simulink model "WSCC_Indian_400kV_test1"  (R2021b)
settings: Solver=FixedStepDiscrete  StartTime=0.0  StopTime=1  FixedStep=5e-7  RelTol=1e-3
undefined symbols (not defined in the file or in its folder): D1, Delta
libraries: spsPowerPositiveSequenceLib x24, spsThreePhaseVIMeasurementLib x21, spsFourierLib x18, spsThreePhaseBreakerLib x12, spsDistributedParametersLineLib x12, spsLoadFlowBusLib x9, spsRMSLib x6, spsThreePhaseParallelRLCLoadLib x6, spsSynchronousMachinepuStandardLib x4, spsExcitationSystemLib x3, spsMultiBandPowerSystemStabilizerLib x3, spsSteamTurbineandGovernorLib x3
(part 1 of 2)
settings Model: Creator=MARI  LastModifiedBy=DELL
settings SolverCC: AlgebraicLoopSolver=TrustRegion
settings DataIOCC: SignalLogging=off  DSMLogging=off
settings DebuggingCC: UnconnectedInputMsg=none  UnconnectedOutputMsg=none  UnconnectedLineMsg=none  SFMachineParentedDataDiag=warning  ArithmeticOperatorsInVariantConditions=warning
settings SFSimCC: SimUseLocalCustomCode=off  CustomCodeUndefinedFunction=UseInterfaceOnly
settings RTWCC: RTWUseLocalCustomCode=off

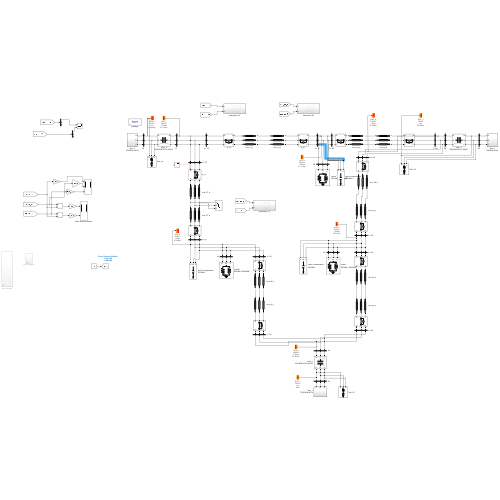
[thumbnail: Simulink's stored preview of the top-level diagram]
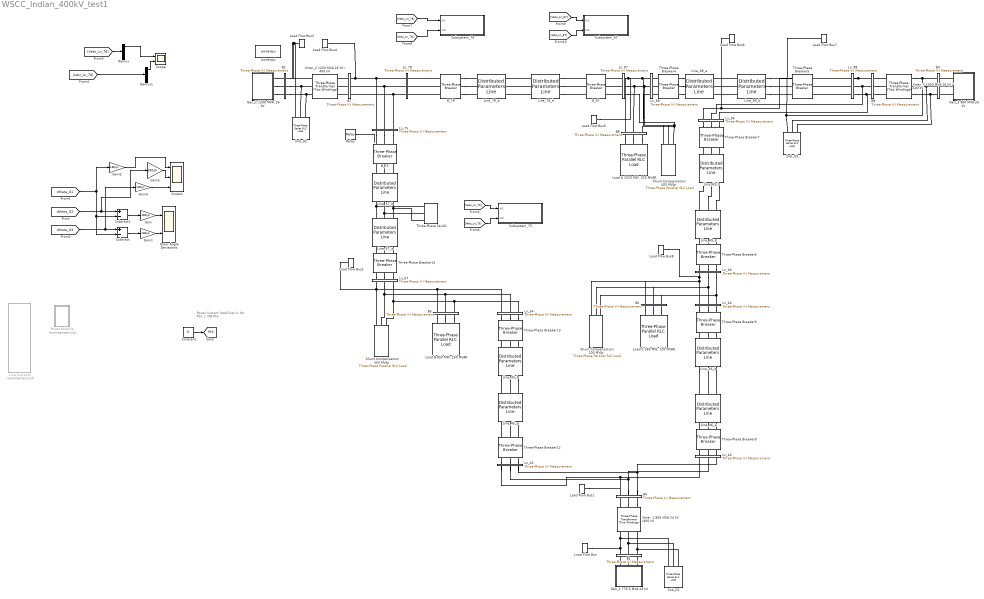
== system WSCC_Indian_400kV_test1 ==
  note: Power System Stabilizer
      | 0: No PSS
      | 1: MB-PSS
  B1 : spsThreePhaseVIMeasurementLib/Three-Phase V-I Measurement  VoltageMeasurement=phase-to-ground  SetLabelV=on  LabelV=Vabc_G1  Vpu=off  VpuLL=off  CurrentMeasurement=yes  SetLabelI=on  LabelI=Iabc_G1  Ipu=off  Pbase=100e6  Vbase=500e3  OutputType=Complex  PhasorSimulation=off  PSBequivalent=0
  B2 : spsThreePhaseVIMeasurementLib/Three-Phase V-I Measurement  VoltageMeasurement=phase-to-ground  SetLabelV=on  LabelV=Vabc_G2  Vpu=off  VpuLL=off  CurrentMeasurement=yes  SetLabelI=on  LabelI=Iabc_G2  Ipu=off  Pbase=100e6  Vbase=500e3  OutputType=Complex  PhasorSimulation=off  PSBequivalent=0
  B3 : spsThreePhaseVIMeasurementLib/Three-Phase V-I Measurement  VoltageMeasurement=phase-to-ground  SetLabelV=on  LabelV=Vabc_G3  Vpu=off  VpuLL=off  CurrentMeasurement=yes  SetLabelI=on  LabelI=Iabc_G3  Ipu=off  Pbase=100e6  Vbase=500e3  OutputType=Complex  PhasorSimulation=off  PSBequivalent=0
  B4 : spsThreePhaseVIMeasurementLib/Three-Phase V-I Measurement  VoltageMeasurement=phase-to-ground  SetLabelV=on  LabelV=Vabc_X1  Vpu=off  VpuLL=off  CurrentMeasurement=yes  SetLabelI=on  LabelI=Iabc_X1  Ipu=off  Pbase=100e6  Vbase=500e3  OutputType=Complex  PhasorSimulation=off  PSBequivalent=0
  B5 : spsThreePhaseVIMeasurementLib/Three-Phase V-I Measurement  VoltageMeasurement=phase-to-ground  SetLabelV=on  LabelV=Vabc_Ld_B  Vpu=off  VpuLL=off  CurrentMeasurement=yes  SetLabelI=on  LabelI=Iabc_Ld_B  Ipu=off  Pbase=100e6  Vbase=500e3  OutputType=Complex  PhasorSimulation=off  PSBequivalent=0
  B6 : spsThreePhaseVIMeasurementLib/Three-Phase V-I Measurement  VoltageMeasurement=phase-to-ground  SetLabelV=on  LabelV=Vabc_Ld_C  Vpu=off  VpuLL=off  CurrentMeasurement=yes  SetLabelI=on  LabelI=Iabc_Ld_C  Ipu=off  Pbase=100e6  Vbase=500e3  OutputType=Complex  PhasorSimulation=off  PSBequivalent=0
  B7 : spsThreePhaseVIMeasurementLib/Three-Phase V-I Measurement  VoltageMeasurement=phase-to-ground  SetLabelV=on  LabelV=Vabc_X2  Vpu=off  VpuLL=off  CurrentMeasurement=yes  SetLabelI=on  LabelI=Iabc_X2  Ipu=off  Pbase=100e6  Vbase=500e3  OutputType=Complex  PhasorSimulation=off  PSBequivalent=0
  B8 : spsThreePhaseVIMeasurementLib/Three-Phase V-I Measurement  VoltageMeasurement=phase-to-ground  SetLabelV=on  LabelV=Vabc_Ld_A  Vpu=off  VpuLL=off  CurrentMeasurement=yes  SetLabelI=on  LabelI=Iabc_Ld_A  Ipu=off  Pbase=100e6  Vbase=500e3  OutputType=Complex  PhasorSimulation=off  PSBequivalent=0
  B9 : spsThreePhaseVIMeasurementLib/Three-Phase V-I Measurement  VoltageMeasurement=phase-to-ground  SetLabelV=on  LabelV=Vabc_X3  Vpu=off  VpuLL=off  CurrentMeasurement=yes  SetLabelI=on  LabelI=Iabc_X3  Ipu=off  Pbase=100e6  Vbase=500e3  OutputType=Complex  PhasorSimulation=off  PSBequivalent=0
  B_75 : spsThreePhaseBreakerLib/Three-Phase Breaker  InitialState=closed  SwitchA=on  SwitchB=on  SwitchC=on  SwitchTimes=[(0.5+(10/50)) ]  External=off  BreakerResistance=0.01  SnubberResistance=10e6  SnubberCapacitance=inf  Measurements=None
  B_78 : spsThreePhaseBreakerLib/Three-Phase Breaker  InitialState=closed  SwitchA=on  SwitchB=on  SwitchC=on  SwitchTimes=[500 501]  External=off  BreakerResistance=0.01  SnubberResistance=10e6  SnubberCapacitance=inf  Measurements=None
  B_87 : spsThreePhaseBreakerLib/Three-Phase Breaker  InitialState=closed  SwitchA=on  SwitchB=on  SwitchC=on  SwitchTimes=[500 501]  External=off  BreakerResistance=0.01  SnubberResistance=10e6  SnubberCapacitance=inf  Measurements=None
  Constant : Constant  Value=0
  Demux : Demux  Outputs=3
  Demux1 : Demux  Outputs=3
  Gain{,1..4} (5 alike) : Gain  Gain=180/pi
  Gen_1 776.5 MVA 24 kV : Subsystem
  "Gen_2 1200 MVA, 26 kV" : Subsystem
  Gen_3 960 MVA 26 kV : Subsystem
  Line Currents : Subsystem  Commented=on
  Line_45_a : spsDistributedParametersLineLib/Distributed Parameters Line  Phases=3  Length=75  Frequency=50  Resistance=[0.0298 0.1619]  Inductance=[1.0568e-03 3.9470e-03]  Capacitance=[11.0414e-09 7.1301e-09]  x1=[-0.0004 -0.000502771468099836 0 0;-0.00038 -0.000503064432045214 0 0;-0.00036 -0.0005033375358682 0 0;-0.00034 -0.000503590768787121 0 0;-0.00032 -0.000503824120804777 0 0;-0.0003 -0.000504037582708828 0 0;-0.00028 -0.000504231146072164 0 0;-0.00026 -0.000504404803253235 321732.78649115 -262633.17742718;-0.00024 -0.000504558547396353 323376.587232023 -260606.503067403;-0.00022 -0.000504692372431963 325007.621618941 -258569.540409116;-0.0002 -0.00050480627307688 326625.82526146 -256522.369868115;-0.00018 -0.000504900244834504 328231.13427567 -254465.072263188;-0.00016 -0.000504974283994989 329823.485286721 -252397.728812922;-0.00014 -0.000505028387635396 331402.815431322 -250320.421132497;-0.00012 -0.000505062553619807 332969.062360221 -248233.231230462;-0.0001 -0.000505076780599406 334522.164240673 -246136.241505503;-8e-05 -0.000505071068012537 336062.059758874 -244029.534743181;-6e-05 -0.000505045416084724 337588.688122387 -241913.194112673;-4e-05 -0.000504999825828659 339101.989062536 -239787.303163483;-2e-05 -0.000504934299044169 340601.902836794 -237651.945822146]  x2=[-0.0004 -0.000304221159060057 0 0;-0.00038 -0.000305822060913406 0 0;-0.00036 -0.000307410889435441 0 0;-0.00034 -0.000308987581901933 0 0;-0.00032 -0.000310552076067763 0 0;-0.0003 -0.000312104310169381 0 0;-0.00028 -0.000313644222927241 0 0;-0.00026 -0.000315171753548224 311256.788658124 -279965.050017297;-0.00024 -0.000316686841728039 313009.694944229 -278003.855758553;-0.00022 -0.000318189427653596 314750.244143536 -276031.686383603;-0.0002 -0.000319679452005377 316478.367542143 -274048.619750316;-0.00018 -0.000321156855959772 318193.996916697 -272054.734146767;-0.00016 -0.000322621581191402 319897.064537089 -270050.108288147;-0.00014 -0.000324073569875424 321587.503169124 -268034.821313651;-0.00012 -0.00032551276468981 323265.24607718 -266008.952783359;-0.0001 -0.000326939108817612 324930.227026839 -263972.582675092;-8e-05 -0.000328352545949208 326582.380287505 -261925.791381254;-6e-05 -0.00032975302028452 328221.640634996 -259868.659705661;-4e-05 -0.000331140476535219 329847.943354121 -257801.268860349;-2e-05 -0.000332514859926907 331461.224241231 -255723.700462369]  x3=[-0.0004 1.79041224432942e-06 0 0;-0.00038 1.80104414370409e-06 0 0;-0.00036 1.81160494093986e-06 0 0;-0.00034 1.82209421911451e-06 0 0;-0.00032 1.83251156412933e-06 0 0;-0.0003 1.84285656472535e-06 0 0;-0.00028 1.85312881249967e-06 0 0;-0.00026 1.86332790192154e-06 274.200396477289 -531.482257577145;-0.00024 1.87345343034838e-06 277.534330866206 -529.748933487783;-0.00022 1.88350499804164e-06 280.857308674955 -527.994695817602;-0.0002 1.89348220818267e-06 284.169198718062 -526.219613820901;-0.00018 1.90338466688827e-06 287.469870247779 -524.42375757488;-0.00016 1.91321198322634e-06 290.759192959247 -522.607197976866;-0.00014 1.92296376923126e-06 294.037036995635 -520.770006741524;-0.00012 1.93263963991921e-06 297.303272953275 -518.912256398016;-0.0001 1.94223921330338e-06 300.557771886764 -517.034020287146;-8e-05 1.95176211040906e-06 303.800405314056 -515.135372558459;-6e-05 1.96120795528857e-06 307.031045221536 -513.216388167316;-4e-05 1.97057637503614e-06 310.249564069072 -511.277142871936;-2e-05 1.97986699980258e-06 313.45583479505 -509.317713230402]  x4=[-0.0004 -2.83648823554354e-06 0 0;-0.00038 -2.85005809032082e-06 0 0;-0.00036 -2.86351542968476e-06 0 0;-0.00034 -2.87685972236267e-06 0 0;-0.00032 -2.89009044154471e-06 0 0;-0.0003 -2.90320706490475e-06 0 0;-0.00028 -2.91620907462095e-06 0 0;-0.00026 -2.92909595739623e-06 1690.40881793717 -1294.98045174982;-0.00024 -2.94186720447853e-06 1698.51196506254 -1284.33382392094;-0.00022 -2.95452231168089e-06 1706.54805784385 -1273.63649279182;-0.0002 -2.96706077940133e-06 1714.51677902991 -1262.88888067478;-0.00018 -2.97948211264262e-06 1722.41781402926 -1252.09141186715;-0.00016 -2.99178582103179e-06 1730.25085092256 -1241.2445126345;-0.00014 -3.00397141883951e-06 1738.01558047493 -1230.34861119384;-0.00012 -3.01603842499923e-06 1745.71169614815 -1219.4041376967;-0.0001 -3.02798636312623e-06 1753.33889411274 -1208.41152421216;-8e-05 -3.03981476153634e-06 1760.89687325998 -1197.37120470978;-6e-05 -3.05152315326467e-06 1768.38533521381 -1186.28361504246;-4e-05 -3.06311107608395e-06 1775.80398434256 -1175.14919292927;-2e-05 -3.07457807252284e-06 1783.15252777068 -1163.96837793812]  x5=0.000397871322084792  V1=[1.62e-10 4.153e+05 4.153e+05;314.2 314.2 314.2;-0.6943 0.8874 -0.6834]  V2=[8.471e-10 4.186e+05 4.186e+05;314.2 314.2 314.2;-0.039 0.8395 -0.7313]  I1=[7.601e-12 598 598;314.2 314.2 314.2;-1.312 0.4775 -1.093]  I2=[4.421e-12 2129 2129;314.2 314.2 314.2;2.105 0.9183 -0.6525]  nHarmo=1  Measurements=None  Decoupling=off  VsMag0=0  VrMag0=0  VsAngle0=0  VrAngle0=0  IsMag0=0  IrMag0=0  IsAngle0=0  IrAngle0=0
      settings: SourceProductBaseCode=PS
  Line_45_b : spsDistributedParametersLineLib/Distributed Parameters Line  Phases=3  Length=75  Frequency=50  Resistance=[0.0298 0.1619]  Inductance=[1.0568e-03 3.9470e-03]  Capacitance=[11.0414e-09 7.1301e-09]  x1=[-0.0004 -0.000304221158148138 0 0;-0.00038 -0.00030582206004686 0 0;-0.00036 -0.000307410888614303 0 0;-0.00034 -0.000308987581126235 0 0;-0.00032 -0.000310552075337536 0 0;-0.0003 -0.000312104309484653 0 0;-0.00028 -0.000313644222288039 0 0;-0.00026 -0.000315171752954575 311256.788658124 -279965.050017297;-0.00024 -0.000316686841179964 313009.694944229 -278003.855758553;-0.00022 -0.000318189427151118 314750.244143536 -276031.686383603;-0.0002 -0.000319679451548516 316478.367542143 -274048.619750316;-0.00018 -0.000321156855548546 318193.996916697 -272054.734146767;-0.00016 -0.000322621580825827 319897.064537089 -270050.108288147;-0.00014 -0.000324073569555514 321587.503169124 -268034.821313651;-0.00012 -0.000325512764415577 323265.24607718 -266008.952783359;-0.0001 -0.000326939108589069 324930.227026839 -263972.582675092;-8e-05 -0.000328352545766363 326582.380287505 -261925.791381254;-6e-05 -0.00032975302014738 328221.640634996 -259868.659705661;-4e-05 -0.000331140476443789 329847.943354121 -257801.268860349;-2e-05 -0.000332514859881191 331461.224241231 -255723.700462369]  x2=[-0.0004 -0.000101444730046378 0 0;-0.00038 -0.000104324693694344 0 0;-0.00036 -0.000107200538782035 0 0;-0.00034 -0.000110072151776012 0 0;-0.00032 -0.00011293941930991 0 0;-0.0003 -0.000115802228188917 0 0;-0.00028 -0.000118660465394241 0 0;-0.00026 -0.00012151401808757 298928.168184214 -295303.504320511;-0.00024 -0.00012436277361553 300777.691716674 -293419.469778965;-0.00022 -0.000127206619514131 302615.341060879 -291523.851539167;-0.0002 -0.000130045443513206 304441.04366958 -289616.724436879;-0.00018 -0.000132879133540845 306254.727467163 -287698.163762213;-0.00016 -0.000135707577727817 308056.320852498 -285768.24525666;-0.00014 -0.000138530664411989 309845.752701762 -283827.045110098;-0.00012 -0.000141348282142733 311622.952371251 -281874.639957785;-0.0001 -0.000144160319685325 313387.849700164 -279911.106877333;-8e-05 -0.000146966666025337 315140.375013377 -277936.523385665;-6e-05 -0.000149767210373022 316880.459124191 -275950.967435959;-4e-05 -0.000152561842167684 318608.033337065 -273954.517414561;-2e-05 -0.000155350451082045 320323.029450327 -271947.252137902]  x3=[-0.0004 2.02866006741614e-06 0 0;-0.00038 2.03797882812101e-06 0 0;-0.00036 2.04721713291132e-06 0 0;-0.00034 2.05637461707463e-06 0 0;-0.00032 2.06545091908913e-06 0 0;-0.0003 2.07444568063796e-06 0 0;-0.00028 2.08335854662334e-06 0 0;-0.00026 2.09218916518058e-06 310.890797679776 -505.121481452329;-0.00024 2.10093718769198e-06 314.058378790467 -503.15814394328;-0.00022 2.10960226880059e-06 317.213561414117 -501.174942612253;-0.0002 2.11818406642385e-06 320.356220989519 -499.17195575264;-0.00018 2.12668224176708e-06 323.486233449855 -497.149262438933;-0.00016 2.13509645933686e-06 326.60347522759 -495.106942523601;-0.00014 2.1434263869543e-06 329.707823259359 -493.045076633937;-0.00012 2.15167169576812e-06 332.799154990816 -490.963746168876;-0.0001 2.15983206026764e-06 335.877348381477 -488.863033295781;-8e-05 2.16790715829565e-06 338.942281909537 -486.743020947199;-6e-05 2.1758966710611e-06 341.993834576671 -484.603792817588;-4e-05 2.18380028315171e-06 345.031885912802 -482.44543336001;-2e-05 2.1916176825464e-06 348.056315980867 -480.268027782803]  x4=[-0.0004 -2.50765540919302e-06 0 0;-0.00038 -2.52313716712917e-06 0 0;-0.00036 -2.53851931593026e-06 0 0;-0.00034 -2.5538012483354e-06 0 0;-0.00032 -2.56898236104007e-06 0 0;-0.0003 -2.58406205471992e-06 0 0;-0.00028 -2.59903973405448e-06 0 0;-0.00026 -2.6139148077506e-06 1576.16809573043 -1423.41445174119;-0.00024 -2.62868668856586e-06 1585.08046857421 -1413.48308229739;-0.00022 -2.64335479333168e-06 1593.93026515519 -1403.49591096177;-0.0002 -2.65791854297641e-06 1602.71713609855 -1393.45333201075;-0.00018 -2.67237736254814e-06 1611.44073451366 -1383.35574190816;-0.00016 -2.68673068123745e-06 1620.1007160078 -1373.20353928956;-0.00014 -2.70097793239988e-06 1628.69673869974 -1362.99712494653;-0.00012 -2.71511855357836e-06 1637.2284632332 -1352.73690181084;-0.0001 -2.72915198652537e-06 1645.69555279032 -1342.42327493852;-8e-05 -2.74307767722501e-06 1654.0976731049 -1332.0566514939;-6e-05 -2.75689507591485e-06 1662.43449247561 -1321.63744073352;-4e-05 -2.77060363710765e-06 1670.7056817791 -1311.16605398999;-2e-05 -2.7842028196129e-06 1678.91091448298 -1300.64290465573]  x5=0.000397871322084792  V1=[8.377e-10 4.186e+05 4.186e+05;314.2 314.2 314.2;-0.02057 0.8395 -0.7313]  V2=[8.866e-10 4.202e+05 4.202e+05;314.2 314.2 314.2;-0.5299 0.7927 -0.7781]  I1=[5.663e-12 593.1 593.1;314.2 314.2 314.2;-2.774 0.5529 -1.018]  I2=[8.582e-12 2124 2124;314.2 314.2 314.2;-0.07241 0.8375 -0.7333]  nHarmo=1  Measurements=None  Decoupling=off  VsMag0=0  VrMag0=0  VsAngle0=0  VrAngle0=0  IsMag0=0  IrMag0=0  IsAngle0=0  IrAngle0=0
      settings: SourceProductBaseCode=PS
  Line_46_a : spsDistributedParametersLineLib/Distributed Parameters Line  Phases=3  Length=90  Frequency=50  Resistance=[0.0298 0.1619]  Inductance=[1.0568e-03 3.9470e-03]  Capacitance=[11.0414e-09 7.1301e-09]  x1=[-0.00048 -0.000501560047261789 302830.615039264 -284229.099929761;-0.00046 -0.000501933189116344 304610.479429935 -282320.765073419;-0.00044 -0.000502286515508039 306378.318320455 -280401.284676681;-0.00042 -0.000502620012488154 308134.061919571 -278470.734517349;-0.0004 -0.0005029336668908 309877.640913533 -276529.190810236;-0.00038 -0.000503227466333437 311608.986468827 -274576.730204164;-0.00036 -0.000503501399217366 313328.030234895 -272613.429778934;-0.00034 -0.000503755454728187 315034.704346833 -270639.367042285;-0.00032 -0.000503989622836223 316728.941428069 -268654.619926835;-0.0003 -0.000504203894296918 318410.674593024 -266659.266787;-0.00028 -0.000504398260651201 320079.837449753 -264653.386395906;-0.00026 -0.000504572714225822 321736.364102564 -262637.057942276;-0.00024 -0.000504727248133652 323380.189154621 -260610.361027305;-0.00022 -0.000504861856273957 325011.247710526 -258573.375661518;-0.0002 -0.000504976533332639 326629.475378879 -256526.182261608;-0.00018 -0.000505071274782443 328234.808274824 -254468.861647265;-0.00016 -0.000505146076883138 329827.183022566 -252401.495037985;-0.00014 -0.000505200936681668 331406.536757877 -250324.164049862;-0.00012 -0.000505235852012259 332972.807130575 -248236.950692365;-0.0001 -0.000505250821496516 334525.932306989 -246139.937365105;-8e-05 -0.000505245844543468 336065.850972396 -244033.206854577;-6e-05 -0.000505220921349597 337592.502333443 -241916.842330894;-4e-05 -0.000505176052898827 339105.826120549 -239790.927344503;-2e-05 -0.000505111240962489 340605.762590282 -237655.545822889]  x2=[-0.00048 -0.000411402495441232 301814.120064113 -295110.747830471;-0.00046 -0.000412537416535352 303662.375446272 -293208.584902774;-0.00044 -0.000413656051358644 305498.642757803 -291294.846602198;-0.00042 -0.000414758355749321 307322.849506015 -289369.608479855;-0.0004 -0.000415844286190294 309134.923674349 -287432.94654085;-0.00038 -0.000416913799810887 310934.79372522 -285484.937241279;-0.00036 -0.000417966854388534 312722.388602841 -283525.657485215;-0.00034 -0.000419003408350444 314497.637736026 -281555.184621666;-0.00032 -0.00042002342077524 316260.47104098 -279573.596441529;-0.0003 -0.00042102685139458 318010.818924061 -277580.97117451;-0.00028 -0.000422013660594741 319748.612284534 -275577.387486045;-0.00026 -0.000422983809418184 321473.78251729 -273562.924474185;-0.00024 -0.000423937259565096 323186.261515564 -271537.661666482;-0.00022 -0.000424873973394897 324885.981673617 -269501.679016844;-0.0002 -0.000425793913927729 326572.875889407 -267455.056902378;-0.00018 -0.000426697044845915 328246.87756724 -265397.876120223;-0.00016 -0.000427583330495393 329907.920620395 -263330.217884352;-0.00014 -0.000428452735887123 331555.939473736 -261252.163822373;-0.00012 -0.000429305226698468 333190.869066302 -259163.795972301;-0.0001 -0.000430140769274552 334812.644853872 -257065.196779324;-8e-05 -0.000430959330629584 336421.202811513 -254956.449092544;-6e-05 -0.000431760878448163 338016.479436113 -252837.636161709;-4e-05 -0.000432545381086555 339598.411748882 -250708.841633926;-2e-05 -0.000433312807573937 341166.93729784 -248570.149550358]  x3=[-0.00048 5.0379673701657e-07 565.011346386232 -958.487842072313;-0.00046 5.07060669066249e-07 571.022475906846 -954.918889885602;-0.00044 5.1030458322894e-07 577.011062437859 -951.312239136202;-0.00042 5.13528351440467e-07 582.976869560128 -947.668032208508;-0.0004 5.16731846431981e-07 588.919661753803 -943.98641296957;-0.00038 5.19914941734984e-07 594.839204407624 -940.267526763412;-0.00036 5.23077511686324e-07 600.735263828183 -936.511520405293;-0.00034 5.26219431433155e-07 606.60760724915 -932.718542175913;-0.00032 5.29340576937865e-07 612.456002840461 -928.888741815558;-0.0003 5.32440824982974e-07 618.280219717472 -925.022270518188;-0.00028 5.35520053175997e-07 624.080027950074 -921.11928092547;-0.00026 5.38578139954278e-07 629.855198571769 -917.17992712075;-0.00024 5.41614964589788e-07 635.605503588709 -913.20436462297;-0.00022 5.44630407193888e-07 641.330715988698 -909.192750380532;-0.0002 5.47624348722069e-07 647.030609750155 -905.145242765096;-0.00018 5.50596670978646e-07 652.704959851032 -901.062001565333;-0.00016 5.53547256621425e-07 658.353542277704 -896.943187980613;-0.00014 5.56475989166337e-07 663.976134033809 -892.788964614644;-0.00012 5.59382752992036e-07 669.572513149051 -888.599495469052;-0.0001 5.62267433344464e-07 675.142458687966 -884.374945936905;-8e-05 5.6512991634138e-07 680.685750758641 -880.115482796184;-6e-05 5.67970088976855e-07 686.202170521397 -875.821274203202;-4e-05 5.70787839125739e-07 691.691500197427 -871.492489685961;-2e-05 5.73583055548079e-07 697.153523077395 -867.129300137461]  x4=[-0.00048 -1.68866517687854e-06 1286.6185695547 -996.034783563132;-0.00046 -1.69450056563087e-06 1292.85137214031 -987.93112610945;-0.00044 -1.70026905840232e-06 1299.03313516747 -979.788466826519;-0.00042 -1.70597042746267e-06 1305.16361459075 -971.607127172583;-0.0004 -1.71160444773163e-06 1311.24256838933 -963.387430132925;-0.00038 -1.71717089678774e-06 1317.26975657651 -955.129700207109;-0.00036 -1.7226695548771e-06 1323.24494120923 -946.834263396172;-0.00034 -1.72810020492212e-06 1329.16788639743 -938.501447189757;-0.00032 -1.73346263253004e-06 1335.03835831338 -930.131580553178;-0.0003 -1.73875662600138e-06 1340.85612520089 -921.72499391444;-0.00028 -1.74398197633836e-06 1346.62095738449 -913.282019151187;-0.00026 -1.74913847725309e-06 1352.33262727848 -904.802989577608;-0.00024 -1.75422592517574e-06 1357.99090939591 -896.288239931271;-0.00022 -1.75924411926258e-06 1363.59558035749 -887.738106359913;-0.0002 -1.7641928614039e-06 1369.1464189004 -879.152926408167;-0.00018 -1.76907195623183e-06 1374.64320588705 -870.533039004238;-0.00016 -1.77388121112807e-06 1380.0857243137 -861.87878444652;-0.00014 -1.77862043623147e-06 1385.47375931904 -853.190504390164;-0.00012 -1.78328944444552e-06 1390.80709819267 -844.468541833592;-0.0001 -1.7878880514458e-06 1396.08553038351 -835.71324110495;-8e-05 -1.79241607568715e-06 1401.30884750809 -826.924947848519;-6e-05 -1.79687333841095e-06 1406.47684335879 -818.104009011069;-4e-05 -1.80125966365208e-06 1411.589313912 -809.250772828162;-2e-05 -1.80557487824595e-06 1416.64605733611 -800.365588810403]  x5=0.00047744558650175  V1=[2.78e-10 4.153e+05 4.153e+05;314.2 314.2 314.2;2.169 0.8713 -0.6995]  V2=[5.247e-10 4.221e+05 4.221e+05;314.2 314.2 314.2;2.009 0.8508 -0.72]  I1=[2.389e-12 1113 1113;314.2 314.2 314.2;0.1121 0.5869 -0.9839]  I2=[3.387e-12 1627 1627;314.2 314.2 314.2;-2.917 0.9662 -0.6046]  nHarmo=1  Measurements=None  Decoupling=off  VsMag0=0  VrMag0=0  VsAngle0=0  VrAngle0=0  IsMag0=0  IrMag0=0  IsAngle0=0  IrAngle0=0
      settings: SourceProductBaseCode=PS
  Line_46_b : spsDistributedParametersLineLib/Distributed Parameters Line  Phases=3  Length=30  Frequency=50  Resistance=[0.0298 0.1619]  Inductance=[1.0568e-03 3.9470e-03]  Capacitance=[11.0414e-09 7.1301e-09]  x1=[-0.00016 -0.000427583129495438 0 0;-0.00014 -0.000428452536338134 0 0;-0.00012 -0.000429305028608323 333190.869066302 -259163.795972301;-0.0001 -0.00043014057265107 334812.644853872 -257065.196779324;-8e-05 -0.000430959135480528 336421.202811513 -254956.449092544;-6e-05 -0.000431760684781237 338016.479436113 -252837.63616171;-4e-05 -0.000432545188909404 339598.411748882 -250708.841633927;-2e-05 -0.000433312616894149 341166.93729784 -248570.149550358]  x2=[-0.00016 -0.00039957058900375 0 0;-0.00014 -0.000400706221820434 0 0;-0.00012 -0.0004018260354416 332620.383400947 -262211.604993758;-0.0001 -0.000402929985658923 334261.320285234 -260116.530054087;-8e-05 -0.000404018028890339 335889.061104942 -258011.1861592;-6e-05 -0.000405090122181764 337503.541599652 -255895.656424469;-4e-05 -0.000406146223208791 339104.698032439 -253770.024367386;-2e-05 -0.000407186290278359 340692.467192387 -251634.373904265]  x3=[-0.00016 6.43590219094434e-07 0 0;-0.00014 6.46038592009079e-07 0 0;-0.00012 6.48461460426307e-07 752.921648469987 -823.661569175122;-0.0001 6.5085872869542e-07 758.081933342957 -818.914603332279;-8e-05 6.53230302176374e-07 763.212290439242 -814.135308143103;-6e-05 6.55576087243507e-07 768.312517221129 -809.323872285985;-4e-05 6.57895991289242e-07 773.382412340399 -804.480485708173;-2e-05 6.60189922727739e-07 778.421775646271 -799.605339618277]  x4=[-0.00016 -1.73911521278104e-06 0 0;-0.00014 -1.74441958433319e-06 0 0;-0.00012 -1.74965508918707e-06 1367.4500122605 -892.543346672269;-0.0001 -1.75482152065392e-06 1373.03096659633 -883.933853984479;-8e-05 -1.75991867477187e-06 1378.5577160206 -875.289465101671;-6e-05 -1.76494635031401e-06 1384.03004234671 -866.610521289516;-4e-05 -1.7699043487963e-06 1389.44772953659 -857.897365177856;-2e-05 -1.77479247448547e-06 1394.81056370922 -849.150340747174]  x5=0.000159148528833917  V1=[5.267e-10 4.221e+05 4.221e+05;314.2 314.2 314.2;2.115 0.9152 -0.6556]  V2=[4.511e-10 4.235e+05 4.235e+05;314.2 314.2 314.2;1.521 0.9087 -0.6621]  I1=[7.622e-12 1116 1116;314.2 314.2 314.2;-1.047 0.7461 -0.8247]  I2=[9.859e-12 1633 1633;314.2 314.2 314.2;1.521 0.998 -0.5728]  nHarmo=1  Measurements=None  Decoupling=off  VsMag0=0  VrMag0=0  VsAngle0=0  VrAngle0=0  IsMag0=0  IrMag0=0  IsAngle0=0  IrAngle0=0
      settings: SourceProductBaseCode=PS
  Line_57_a : spsDistributedParametersLineLib/Distributed Parameters Line  Phases=3  Length=30  Frequency=50  Resistance=[0.0298 0.1619]  Inductance=[1.0568e-03 3.9470e-03]  Capacitance=[11.0414e-09 7.1301e-09]  x1=[-0.00016 -0.000135668678046725 0 0;-0.00014 -0.000138491677767821 0 0;-0.00012 -0.000141309210074614 311628.254179597 -281875.871303439;-0.0001 -0.000144121163735754 313393.159140047 -279912.30488651;-8e-05 -0.000146927427740124 315145.69187519 -277937.68801107;-6e-05 -0.000149727891301228 316885.783198034 -275952.098631613;-4e-05 -0.000152522443861558 318613.364412752 -273955.615135808;-2e-05 -0.000155310975096964 320328.367317397 -271948.316341405]  x2=[-0.00016 -0.000140869936296788 0 0;-0.00014 -0.000144023169049062 0 0;-0.00012 -0.000147170716013229 318212.683484871 -270595.610200224;-0.0001 -0.000150312452929524 319906.582990812 -268590.894991504;-8e-05 -0.000153448255767554 321587.853132623 -266575.57627415;-6e-05 -0.000156578000731192 323256.42753664 -264549.733609496;-4e-05 -0.000159701564263466 324912.240330401 -262513.446974341;-2e-05 -0.000162818823051435 326555.226145253 -260466.796757794]  x3=[-0.00016 1.20141200238615e-06 0 0;-0.00014 1.19558293287482e-06 0 0;-0.00012 1.18970666379647e-06 2171.30028900687 -1479.61599878337;-0.0001 1.18378342713614e-06 2180.55398293649 -1465.94420267311;-8e-05 1.17781345673306e-06 2189.72159232857 -1452.21453359583;-6e-05 1.17179698827146e-06 2198.80275526158 -1438.42753357535;-4e-05 1.16573425927119e-06 2207.79711322677 -1424.58374689883;-2e-05 1.15962550907842e-06 2216.70431114229 -1410.68372009526]  x4=[-0.00016 -1.53938439904887e-06 0 0;-0.00014 -1.54160729350236e-06 0 0;-0.00012 -1.54376932793955e-06 -168.560626532057 -335.015068612418;-0.0001 -1.54587041700703e-06 -166.452331634511 -336.067560964944;-8e-05 -1.5479104777574e-06 -164.337465483925 -337.106785945602;-6e-05 -1.54988942965256e-06 -162.216111571592 -338.132702527571;-4e-05 -1.55180719456688e-06 -160.088353644933 -339.145270209421;-2e-05 -1.55366369679026e-06 -157.954275704187 -340.144449016711]  x5=0.000159148528833917  V1=[8.847e-10 4.202e+05 4.202e+05;314.2 314.2 314.2;0.04885 0.841 -0.7298]  V2=[4.139e-10 4.177e+05 4.177e+05;314.2 314.2 314.2;-0.2267 0.8716 -0.6992]  I1=[1.496e-11 2628 2628;314.2 314.2 314.2;1.536 0.9781 -0.5927]  I2=[1.402e-11 375 375;314.2 314.2 314.2;-1.159 -0.4607 -2.031]  nHarmo=1  Measurements=None  Decoupling=off  VsMag0=0  VrMag0=0  VsAngle0=0  VrAngle0=0  IsMag0=0  IrMag0=0  IsAngle0=0  IrAngle0=0
      settings: SourceProductBaseCode=PS
  Line_57_b : spsDistributedParametersLineLib/Distributed Parameters Line  Phases=3  Length=90  Frequency=50  Resistance=[0.0298 0.1619]  Inductance=[1.0568e-03 3.9470e-03]  Capacitance=[11.0414e-09 7.1301e-09]  x1=[-0.00048 -8.97471686358994e-05 285641.466355405 -304779.152094545;-0.00046 -9.29743066059261e-05 287550.789221277 -302978.412940509;-0.00044 -9.61977741095254e-05 289448.760074357 -301165.712717512;-0.00042 -9.94174438897199e-05 291335.303986004 -299341.122987855;-0.0004 -0.00010263318883946 293210.346478695 -297504.715783217;-0.00038 -0.00010584488200664 295073.813528965 -295656.563601809;-0.00036 -0.000109052396599114 296925.631570323 -293796.739405516;-0.00034 -0.000112255605989698 298765.727496165 -291925.316617011;-0.00032 -0.000115454383721171 300594.028662655 -290042.369116863;-0.0003 -0.000118648603511263 302410.462891592 -288147.971240613;-0.00028 -0.000121838139257648 304214.958473264 -286242.197775848;-0.00026 -0.000125022865042915 306007.444169275 -284325.12395924;-0.00024 -0.000128202655139543 307787.849215359 -282396.82547358;-0.00022 -0.000131377384014865 309556.103324173 -280457.378444791;-0.0002 -0.00013454692633602 311312.136688073 -278506.859438921;-0.00018 -0.000137711156974905 313055.879981868 -276545.345459121;-0.00016 -0.000140869951013111 314787.264365559 -274572.913942604;-0.00014 -0.000144023183746859 316506.221487054 -272589.642757588;-0.00012 -0.000147170730691921 318212.683484871 -270595.610200224;-0.0001 -0.000150312467588531 319906.582990812 -268590.894991504;-8e-05 -0.000153448270406297 321587.853132623 -266575.57627415;-6e-05 -0.000156578015349093 323256.42753664 -264549.733609496;-4e-05 -0.000159701578859947 324912.240330401 -262513.446974341;-2e-05 -0.000162818837625921 326555.226145253 -260466.796757794]  x2=[-0.00048 -8.92494800863178e-05 307455.375756809 -271363.243171537;-0.00046 -9.34197076148414e-05 309154.311010086 -269426.102052493;-0.00044 -9.75862470932684e-05 310841.041380521 -267478.324452271;-0.00042 -0.000101748934033755 312515.500278888 -265519.987265796;-0.0004 -0.000105907604100547 314177.621600416 -263551.167804866;-0.00038 -0.000110062093116473 315827.339727402 -261571.943795104;-0.00036 -0.000114212237069419 317464.589531798 -259582.393372883;-0.00034 -0.000118357872118808 319089.306377786 -257582.595082249;-0.00032 -0.000122498834602067 320701.426124326 -255572.627871812;-0.0003 -0.000126634961041088 322300.885127692 -253552.571091638;-0.00028 -0.00013076608814868 323887.620243981 -251522.504490109;-0.00026 -0.00013489205283502 325461.568831606 -249482.508210777;-0.00024 -0.000139012692214085 327022.668753774 -247432.662789204;-0.00022 -0.000143127843610091 328570.858380932 -245373.049149777;-0.0002 -0.000147237344563904 330106.076593204 -243303.748602515;-0.00018 -0.000151341032839465 331628.262782805 -241224.842839861;-0.00016 -0.000155438746430187 333137.35685643 -239136.413933455;-0.00014 -0.000159530323565353 334633.299237628 -237038.544330894;-0.00012 -0.000163615602716505 336116.030869156 -234931.316852478;-0.0001 -0.000167694422603816 337585.493215309 -232814.814687939;-8e-05 -0.000171766622202462 339041.628264228 -230689.121393159;-6e-05 -0.000175832040748975 340484.378530196 -228554.32088687;-4e-05 -0.000179890517747591 341913.687055902 -226410.49744734;-2e-05 -0.000183941892976589 343329.497414693 -224257.735709047]  x3=[-0.00048 1.24767069649791e-06 2040.92110898181 -1646.29998636621;-0.00046 1.24226729905328e-06 2051.22467659665 -1633.44409817671;-0.00044 1.23681485902278e-06 2061.44726537352 -1620.52372441112;-0.00042 1.23131359165941e-06 2071.58847174212 -1607.53937514367;-0.0004 1.22576371414379e-06 2081.64789534498 -1594.49156297423;-0.00038 1.22016544557558e-06 2091.62513905329 -1581.3808030081;-0.00036 1.21451900696483e-06 2101.51980898254 -1568.20761283562;-0.00034 1.20882462122328e-06 2111.33151450811 -1554.97251251179;-0.00032 1.20308251315553e-06 2121.05986828067 -1541.67602453571;-0.0003 1.19729290945016e-06 2130.70448624146 -1528.31867382994;-0.00028 1.19145603867082e-06 2140.26498763749 -1514.90098771984;-0.00026 1.18557213124717e-06 2149.74099503653 -1501.42349591267;-0.00024 1.17964141946581e-06 2159.13213434202 -1487.88673047672;-0.00022 1.17366413746107e-06 2168.43803480788 -1474.29122582033;-0.0002 1.16764052120583e-06 2177.65832905309 -1460.63751867074;-0.00018 1.16157080850212e-06 2186.79265307621 -1446.92614805291;-0.00016 1.15545523897183e-06 2195.84064626978 -1433.1576552683;-0.00014 1.14929405404715e-06 2204.80195143452 -1419.33258387342;-0.00012 1.14308749696113e-06 2213.67621479344 -1405.45147965841;-0.0001 1.13683581273801e-06 2222.46308600582 -1391.5148906255;-8e-05 1.13053924818358e-06 2231.16221818103 -1377.52336696737;-6e-05 1.12419805187542e-06 2239.77326789223 -1363.47746104541;-4e-05 1.11781247415311e-06 2248.29589518992 -1349.37772736793;-2e-05 1.11138276710832e-06 2256.72976361536 -1335.22472256828]  x4=[-0.00048 -1.36694435731923e-06 -225.878466359927 -296.158334271337;-0.00046 -1.37145304467626e-06 -224.013180387174 -297.571725393646;-0.00044 -1.37590758941539e-06 -222.139050757631 -298.973368893762;-0.00042 -1.38030781567882e-06 -220.256151458727 -300.363209437197;-0.0004 -1.38465354975315e-06 -218.364556824102 -301.741192155429;-0.00038 -1.38894462007625e-06 -216.464341530674 -303.107262648057;-0.00036 -1.393180857244e-06 -214.555580595689 -304.461366984959;-0.00034 -1.39736209401701e-06 -212.638349373759 -305.803451708414;-0.00032 -1.40148816532722e-06 -210.712723553892 -307.133463835215;-0.0003 -1.40555890828439e-06 -208.778779156497 -308.451350858761;-0.00028 -1.40957416218257e-06 -206.836592530387 -309.757060751128;-0.00026 -1.4135337685064e-06 -204.886240349765 -311.050541965125;-0.00024 -1.4174375709374e-06 -202.927799611195 -312.331743436329;-0.00022 -1.42128541536015e-06 -200.961347630565 -313.600614585101;-0.0002 -1.42507714986833e-06 -198.986962040031 -314.857105318578;-0.00018 -1.42881262477076e-06 -197.004720784956 -316.101166032659;-0.00016 -1.43249169259728e-06 -195.014702120831 -317.332747613958;-0.00014 -1.43611420810459e-06 -193.016984610185 -318.551801441741;-0.00012 -1.43968002828199e-06 -191.011647119484 -319.758279389851;-0.0001 -1.443189012357e-06 -188.998768816019 -320.952133828605;-8e-05 -1.44664102180094e-06 -186.978429164779 -322.133317626673;-6e-05 -1.45003592033438e-06 -184.950707925314 -323.301784152943;-4e-05 -1.45337357393255e-06 -182.915685148587 -324.457487278355;-2e-05 -1.4566538508306e-06 -180.873441173812 -325.600381377729]  x5=0.00047744558650175  V1=[4.309e-10 4.177e+05 4.177e+05;314.2 314.2 314.2;-0.354 0.8072 -0.7636]  V2=[3.73e-10 4.101e+05 4.101e+05;314.2 314.2 314.2;-0.5088 0.9019 -0.6689]  I1=[1.704e-12 2622 2622;314.2 314.2 314.2;-1.588 0.9462 -0.6246]  I2=[3.147e-12 372.5 372.5;314.2 314.2 314.2;-0.7702 -0.5974 -2.168]  nHarmo=1  Measurements=None  Decoupling=off  VsMag0=0  VrMag0=0  VsAngle0=0  VrAngle0=0  IsMag0=0  IrMag0=0  IsAngle0=0  IrAngle0=0
      settings: SourceProductBaseCode=PS
  Line_69_a : spsDistributedParametersLineLib/Distributed Parameters Line  Phases=3  Length=70  Frequency=50  Resistance=[0.0298 0.1619]  Inductance=[1.0568e-03 3.9470e-03]  Capacitance=[11.0414e-09 7.1301e-09]  x1=[-0.00038 -0.000386033758217423 310120.425886557 -288477.75613815;-0.00036 -0.000387340229756795 311926.84116133 -286523.534066638;-0.00034 -0.000388631409767128 313720.942098517 -284558.000536608;-0.00032 -0.000389907247274848 315502.657870087 -282581.233143958;-0.0003 -0.000391167691912073 317271.918136951 -280593.309928081;-0.00028 -0.000392412693918608 319028.653051744 -278594.30936878;-0.00026 -0.000393642204143905 320772.793261578 -276584.310383175;-0.00024 -0.000394856174049006 322504.269910786 -274563.392322584;-0.00022 -0.000396054555708458 324223.014643634 -272531.634969392;-0.0002 -0.000397237301812204 325928.959607022 -270489.118533901;-0.00018 -0.000398404365667454 327622.037453164 -268435.923651161;-0.00016 -0.000399555701200525 329302.181342247 -266372.131377792;-0.00014 -0.000400691262958662 330969.324945066 -264297.823188778;-0.00012 -0.00040181100611183 332623.402445646 -262213.080974254;-0.0001 -0.000402914886454488 334264.34854384 -260117.987036275;-8e-05 -0.000404002860407329 335892.098457906 -258012.624085561;-6e-05 -0.000405074885019005 337506.587927065 -255897.075238236;-4e-05 -0.000406130917967819 339107.753214035 -253771.424012547;-2e-05 -0.0004071709175634 340695.531107555 -251635.754325564]  x2=[-0.00038 -0.000329380308873669 316155.807890704 -274644.465851235;-0.00036 -0.00033074835335005 317875.187537998 -272652.595012445;-0.00034 -0.000332103340447773 319582.018017178 -270649.96031606;-0.00032 -0.000333445216674267 321276.231945498 -268636.640822668;-0.0003 -0.000334773929054557 322957.762438294 -266612.716014676;-0.00028 -0.000336089425133352 324626.543111621 -264578.265793171;-0.00026 -0.00033739165297712 326282.508084876 -262533.370474762;-0.00024 -0.000338680561176136 327925.591983397 -260478.110788416;-0.00022 -0.000339956098846511 329555.729941045 -258412.567872266;-0.0002 -0.000341218215632201 331172.857602764 -256336.82327041;-0.00018 -0.000342466861706997 332776.911127124 -254250.95892969;-0.00016 -0.00034370198777649 334367.827188839 -252155.057196459;-0.00014 -0.000344923545080018 335945.542981265 -250049.200813328;-0.00012 -0.00034613148539259 337509.996218885 -247933.472915902;-0.0001 -0.00034732576102679 339061.125139764 -245807.957029495;-8e-05 -0.000348506324834662 340598.868507988 -243672.737065836;-6e-05 -0.000349673130209568 342123.165616083 -241527.897319751;-4e-05 -0.00035082613108803 343633.956287407 -239373.522465843;-2e-05 -0.000351965281951547 345131.180878533 -237209.697555141]  x3=[-0.00038 -3.05135110539917e-07 1574.51798971855 -1169.48482061429;-0.00036 -3.0314186349508e-07 1581.83489080406 -1159.56882030653;-0.00034 -3.01136648928534e-07 1589.08934375661 -1149.60704220725;-0.00032 -2.99119546002717e-07 1596.28106218282 -1139.59987959038;-0.0003 -2.97090634349398e-07 1603.40976216597 -1129.54772752158;-0.00028 -2.95049994066536e-07 1610.47516227719 -1119.45098284259;-0.00026 -2.92997705715115e-07 1617.47698358658 -1109.3100441556;-0.00024 -2.90933850315964e-07 1624.41494967422 -1099.12531180751;-0.00022 -2.88858509346562e-07 1631.28878664109 -1088.89718787412;-0.0002 -2.86771764737815e-07 1638.09822311988 -1078.62607614424;-0.00018 -2.84673698870829e-07 1644.84299028569 -1068.31238210377;-0.00016 -2.82564394573651e-07 1651.52282186667 -1057.95651291971;-0.00014 -2.80443935118002e-07 1658.1374541545 -1047.55887742403;-0.00012 -2.78312404215992e-07 1664.68662601482 -1037.11988609757;-0.0001 -2.76169886016811e-07 1671.17007889756 -1026.63995105385;-8e-05 -2.74016465103408e-07 1677.58755684707 -1016.11948602274;-6e-05 -2.71852226489155e-07 1683.93880651234 -1005.55890633421;-4e-05 -2.69677255614485e-07 1690.22357715689 -994.95862890184;-2e-05 -2.67491638343525e-07 1696.44162066874 -984.319072206448]  x4=[-0.00038 -6.12156683714776e-07 371.431970743669 -717.34236974353;-0.00036 -6.1805453436301e-07 375.931798665168 -714.994464994008;-0.00034 -6.23927985276506e-07 380.416785442954 -712.618333487275;-0.00032 -6.29776804581479e-07 384.886754017429 -710.214069028934;-0.0003 -6.35600761376558e-07 389.341527921886 -707.781766535229;-0.00028 -6.41399625741901e-07 393.780931289481 -705.321522029298;-0.00026 -6.47173168748271e-07 398.20478886017 -702.83343263738;-0.00024 -6.52921162466078e-07 402.61292598763 -700.317596584986;-0.00022 -6.5864337997437e-07 407.005168646156 -697.774113193014;-0.0002 -6.64339595369799e-07 411.381343437528 -695.203082873835;-0.00018 -6.70009583775534e-07 415.741277597859 -692.604607127321;-0.00016 -6.75653121350142e-07 420.084799004414 -689.978788536847;-0.00014 -6.81269985296423e-07 424.411736182404 -687.325730765235;-0.00012 -6.86859953870205e-07 428.721918311759 -684.645538550663;-0.0001 -6.92422806389101e-07 433.015175233869 -681.938317702529;-8e-05 -6.97958323241219e-07 437.291337458301 -679.204175097278;-6e-05 -7.03466285893831e-07 441.550236169493 -676.443218674178;-4e-05 -7.08946476902003e-07 445.791703233416 -673.655557431061;-2e-05 -7.14398679917178e-07 450.015571204213 -670.841301420019]  x5=0.000371346567279139  V1=[7.818e-10 4.235e+05 4.235e+05;314.2 314.2 314.2;1.708 0.8658 -0.705]  V2=[9.391e-10 4.188e+05 4.188e+05;314.2 314.2 314.2;1.235 0.8998 -0.671]  I1=[4.724e-12 1961 1961;314.2 314.2 314.2;-0.8175 0.9762 -0.5946]  I2=[5.7e-12 807.8 807.8;314.2 314.2 314.2;1.598 0.522 -1.049]  nHarmo=1  Measurements=None  Decoupling=off  VsMag0=0  VrMag0=0  VsAngle0=0  VrAngle0=0  IsMag0=0  IrMag0=0  IsAngle0=0  IrAngle0=0
      settings: SourceProductBaseCode=PS
  Line_69_b : spsDistributedParametersLineLib/Distributed Parameters Line  Phases=3  Length=70  Frequency=50  Resistance=[0.0298 0.1619]  Inductance=[1.0568e-03 3.9470e-03]  Capacitance=[11.0414e-09 7.1301e-09]  x1=[-0.00038 -0.000329380324621831 316155.807890704 -274644.465851235;-0.00036 -0.000330748369040705 317875.187537998 -272652.595012445;-0.00034 -0.000332103356080301 319582.018017178 -270649.96031606;-0.00032 -0.000333445232248051 321276.231945498 -268636.640822668;-0.0003 -0.000334773944568982 322957.762438294 -266612.716014676;-0.00028 -0.000336089440587806 324626.543111621 -264578.265793171;-0.00026 -0.000337391668370993 326282.508084876 -262533.370474762;-0.00024 -0.00033868057650882 327925.591983397 -260478.110788416;-0.00022 -0.0003399561141174 329555.729941045 -258412.567872266;-0.0002 -0.000341218230840693 331172.857602764 -256336.82327041;-0.00018 -0.000342466876852491 332776.911127124 -254250.95892969;-0.00016 -0.000343702002858389 334367.827188839 -252155.057196459;-0.00014 -0.000344923560097726 335945.542981265 -250049.200813328;-0.00012 -0.000346131500345514 337509.996218885 -247933.472915902;-0.0001 -0.00034732577591434 339061.125139764 -245807.957029495;-8e-05 -0.00034850633965625 340598.868507988 -243672.737065836;-6e-05 -0.000349673144964609 342123.165616083 -241527.897319751;-4e-05 -0.000350826145775941 343633.956287407 -239373.522465843;-2e-05 -0.000351965296571749 345131.180878533 -237209.697555141]  x2=[-0.00038 -0.000268637342747686 320546.923226567 -259102.086729794;-0.00036 -0.000270044699258365 322168.561308959 -257082.932002439;-0.00034 -0.000271441394866708 323777.480728191 -255053.628081124;-0.00032 -0.000272827374433564 325373.61796688 -253014.255079295;-0.0003 -0.000274202583242832 326956.910012261 -250964.893507905;-0.00028 -0.000275566967003624 328527.294358675 -248905.62427224;-0.00026 -0.000276920471852405 330084.709010036 -246836.528668724;-0.00024 -0.000278263044355121 331629.092482281 -244757.688381707;-0.00022 -0.000279594631509309 333160.383805794 -242669.185480246;-0.0002 -0.000280915180746187 334678.522527817 -240571.102414858;-0.00018 -0.000282224639932733 336183.448714832 -238463.52201427;-0.00016 -0.000283522957373741 337675.10295493 -236346.527482148;-0.00014 -0.00028481008181386 339153.426360155 -234220.202393811;-0.00012 -0.000286085962439623 340618.360568832 -232084.630692933;-0.0001 -0.000287350548881446 342069.847747865 -229939.896688228;-8e-05 -0.000288603791215622 343507.830595027 -227786.085050121;-6e-05 -0.00028984563996629 344932.252341216 -225623.280807409;-4e-05 -0.000291076046107387 346343.056752702 -223451.5693439;-2e-05 -0.000292294961064586 347740.188133341 -221271.036395043]  x3=[-0.00038 -2.63173061517856e-07 1662.10103576028 -1049.18720973268;-0.00036 -2.60910938049567e-07 1668.66036024472 -1038.72328248583;-0.00034 -2.58638514264194e-07 1675.15380887533 -1028.21834822237;-0.00032 -2.56355879873139e-07 1681.58112530189 -1017.67282165911;-0.0003 -2.54063124990897e-07 1687.94205578495 -1007.08711911539;-0.00028 -2.51760340131507e-07 1694.23634920587 -996.461658496613;-0.00026 -2.49447616204971e-07 1700.46375707672 -985.796859277776;-0.00024 -2.4712504451367e-07 1706.62403355011 -975.093142486889;-0.00022 -2.44792716748758e-07 1712.71693542885 -964.350930688364;-0.0002 -2.4245072498654e-07 1718.74222217563 -953.570647966329;-0.00018 -2.40099161684843e-07 1724.69965592243 -942.752719907886;-0.00016 -2.37738119679357e-07 1730.58900147998 -931.897573586313;-0.00014 -2.3536769217998e-07 1736.41002634699 -921.005637544198;-0.00012 -2.32987972767129e-07 1742.16250071937 -910.077341776528;-0.0001 -2.30599055388053e-07 1747.84619749928 -899.113117713706;-8e-05 -2.28201034353118e-07 1753.4608923041 -888.113398204525;-6e-05 -2.25794004332091e-07 1759.00636347531 -877.078617499077;-4e-05 -2.23378060350393e-07 1764.48239208718 -866.009211231609;-2e-05 -2.20953297785358e-07 1769.8887619555 -854.905616403327]  x4=[-0.00038 -4.96903443567779e-07 320.936834965027 -744.42938092001;-0.00036 -5.03146786002291e-07 325.607852198414 -742.398210052541;-0.00034 -5.09370265063216e-07 330.266014991327 -740.337730574929;-0.00032 -5.15573635058259e-07 334.911139447473 -738.248023831375;-0.0003 -5.21756651088993e-07 339.543042185294 -736.129172319924;-0.00028 -5.27919069060532e-07 344.1615403452 -733.981259689204;-0.00026 -5.34060645691167e-07 348.766451596792 -731.804370735129;-0.00024 -5.40181138521968e-07 353.357594146059 -729.598591397547;-0.00022 -5.46280305926359e-07 357.934786742554 -727.364008756849;-0.0002 -5.52357907119654e-07 362.497848686551 -725.100711030533;-0.00018 -5.58413702168564e-07 367.046599836178 -722.808787569716;-0.00016 -5.64447452000669e-07 371.580860614527 -720.488328855613;-0.00014 -5.70458918413859e-07 376.100452016748 -718.139426495961;-0.00012 -5.76447864085731e-07 380.60519561711 -715.762173221402;-0.0001 -5.82414052582966e-07 385.09491357605 -713.356662881825;-8e-05 -5.88357248370658e-07 389.56942864719 -710.92299044266;-6e-05 -5.94277216821613e-07 394.028564184337 -708.461251981127;-4e-05 -6.00173724225614e-07 398.472144148455 -705.971544682447;-2e-05 -6.06046537798644e-07 402.899993114615 -703.453966835998]  x5=0.000371346567279139  V1=[9.514e-10 4.188e+05 4.188e+05;314.2 314.2 314.2;1.248 0.8998 -0.671]  V2=[3.385e-10 4.122e+05 4.122e+05;314.2 314.2 314.2;1.899 0.9353 -0.6355]  I1=[9.51e-12 1966 1966;314.2 314.2 314.2;2.181 1.052 -0.5188]  I2=[1.088e-11 810.7 810.7;314.2 314.2 314.2;-0.4113 0.4513 -1.119]  nHarmo=1  Measurements=None  Decoupling=off  VsMag0=0  VrMag0=0  VsAngle0=0  VrAngle0=0  IsMag0=0  IrMag0=0  IsAngle0=0  IrAngle0=0
      settings: SourceProductBaseCode=PS
  Line_78_a : spsDistributedParametersLineLib/Distributed Parameters Line  Phases=3  Length=100  Frequency=50  Resistance=[0.0298 0.1619]  Inductance=[1.0568e-03 3.9470e-03]  Capacitance=[11.0414e-09 7.1301e-09]  x1=[-0.00054 -7.73051971933937e-05 302287.3374613 -277110.315140988;-0.00052 -8.14876133314561e-05 304022.484442419 -275205.532299551;-0.0005 -8.56668124780732e-05 305745.629136421 -273289.884814927;-0.00048 -8.98426296456188e-05 307456.703516506 -271363.448313596;-0.00046 -9.40148999799812e-05 309155.640032386 -269426.298847976;-0.00044 -9.81834587670717e-05 310842.371612957 -267478.512893408;-0.00042 -0.000102348141439327 312516.831668944 -265520.167345148;-0.0004 -0.000106508783582207 314178.954095531 -263551.339515324;-0.00038 -0.000110665220940682 315828.673274971 -261572.107129889;-0.00036 -0.000114817289425725 317465.924079175 -259582.548325547;-0.00034 -0.000118964825120779 319090.641872286 -257582.741646674;-0.00032 -0.000123107664288238 320702.762513226 -255572.766042213;-0.0003 -0.000127245643375906 322302.222358233 -253552.700862559;-0.00028 -0.000131378599023452 323888.958263371 -251522.625856427;-0.00026 -0.000135506368068864 325462.907587024 -249482.621167702;-0.00024 -0.00013962878755489 327024.008192366 -247432.767332276;-0.00022 -0.000143745694735466 328572.198449821 -245373.145274868;-0.0002 -0.000147856927082145 330107.417239486 -243303.836305831;-0.00018 -0.000151962322290515 331629.603953553 -241224.92211794;-0.00016 -0.000156061718286602 333138.698498697 -239136.484783166;-0.00014 -0.000160154953233272 334634.641298448 -237038.606749441;-0.00012 -0.000164241865536617 336117.373295548 -234931.370837396;-0.0001 -0.000168322293852338 337586.835954275 -232814.860237098;-8e-05 -0.000172396077092111 339042.97126276 -230689.15850476;-6e-05 -0.000176463054429951 340485.721735274 -228554.349559447;-4e-05 -0.000180523065308554 341915.030414499 -226410.517679762;-2e-05 -0.000184575949445644 343330.840873775 -224257.747500516]  x2=[-0.00054 1.5529989704267e-05 278360.197725744 -309269.991736583;-0.00052 1.24987452628515e-05 280297.881026936 -307514.913160703;-0.0005 9.46700739237437e-06 282224.498647733 -305747.6944226;-0.00048 6.43489578065547e-06 284139.974528569 -303968.405289046;-0.00046 3.40253013026944e-06 286044.233049736 -302177.116003328;-0.00044 3.70030153819943e-07 287937.199034368 -300373.897282481;-0.00042 -2.66248443078644e-06 289818.79775141 -298558.820314491;-0.0004 -5.69489390506641e-06 291688.954918566 -296731.95675549;-0.00038 -8.72707855468621e-06 293547.596705233 -294893.378726922;-0.00036 -1.17589186741878e-05 295394.649735417 -293043.158812701;-0.00034 -1.47902945717147e-05 297230.041090625 -291181.37005634;-0.00032 -1.78210865737369e-05 299053.698312751 -289308.085958072;-0.0003 -2.08511750297757e-05 300865.549406929 -287423.380471945;-0.00028 -2.38804403171274e-05 302665.522844381 -285527.328002904;-0.00026 -2.69087628455851e-05 304453.547565237 -283620.003403855;-0.00024 -2.99360230621609e-05 306229.552981343 -281701.481972707;-0.00022 -3.29621014558049e-05 307993.468979047 -279771.839449401;-0.0002 -3.59868785621236e-05 309745.225921965 -277831.15201292;-0.00018 -3.9010234968096e-05 311484.754653732 -275879.49627828;-0.00016 -4.20320513167881e-05 313211.986500732 -273916.949293508;-0.00014 -4.50522083120647e-05 314926.853274811 -271943.588536599;-0.00012 -4.80705867232988e-05 316629.287275963 -269959.491912457;-0.0001 -5.10870673900791e-05 318319.22129501 -267964.737749819;-8e-05 -5.41015312269139e-05 319996.58861625 -265959.404798163;-6e-05 -5.71138592279325e-05 321661.323020093 -263943.572224602;-4e-05 -6.01239324715835e-05 323313.358785676 -261917.319610753;-2e-05 -6.3131632125329e-05 324952.630693455 -259880.7269496]  x3=[-0.00054 -1.37951346873867e-06 -99.8081348606585 -314.397358678326;-0.00052 -1.37929607971135e-06 -97.8307507616801 -315.018269151416;-0.0005 -1.37902423843653e-06 -95.8495044721748 -315.626743242637;-0.00048 -1.37869795564605e-06 -93.8644742083534 -316.222756930475;-0.00046 -1.37831724422099e-06 -91.8757383358121 -316.806286685329;-0.00044 -1.37788211919118e-06 -89.8833753664377 -317.377309470444;-0.00042 -1.37739259773462e-06 -87.8874639553089 -317.935802742818;-0.0004 -1.37684869917678e-06 -85.8880828975905 -318.481744454093;-0.00038 -1.37625044498983e-06 -83.8853111254233 -319.015113051425;-0.00036 -1.37559785879183e-06 -81.8792277048076 -319.535887478335;-0.00034 -1.37489096634577e-06 -79.8699118324817 -320.044047175541;-0.00032 -1.37412979555855e-06 -77.8574428327959 -320.539572081767;-0.0003 -1.37331437647989e-06 -75.8419001545803 -321.02244263454;-0.00028 -1.37244474130113e-06 -73.8233633680088 -321.492639770955;-0.00026 -1.37152092435399e-06 -71.8019121614573 -321.950144928436;-0.00024 -1.37054296210918e-06 -69.7776263383583 -322.394940045462;-0.00022 -1.36951089317497e-06 -67.7505858140499 -322.827007562284;-0.0002 -1.36842475829567e-06 -65.7208706126211 -323.246330421615;-0.00018 -1.36728460035004e-06 -63.6885608637527 -323.652892069308;-0.00016 -1.36609046434955e-06 -61.6537367995537 -324.046676455004;-0.00014 -1.36484239743664e-06 -59.6164787513939 -324.427668032771;-0.00012 -1.36354044888288e-06 -57.5768671467328 -324.795851761713;-0.0001 -1.36218467008694e-06 -55.5349825059441 -325.151213106567;-8e-05 -1.36077511457266e-06 -53.4909054391372 -325.493738038275;-6e-05 -1.35931183798688e-06 -51.4447166429747 -325.823413034541;-4e-05 -1.35779489809726e-06 -49.3964968974865 -326.140225080359;-2e-05 -1.35622435478997e-06 -47.3463270628813 -326.444161668532]  x4=[-0.00054 1.42534362990552e-06 1861.82630265685 -1667.64477633131;-0.00052 1.41554230339425e-06 1872.26753025757 -1655.91374866018;-0.0005 1.40568509369665e-06 1882.63484394203 -1644.11734834964;-0.00048 1.39577238995846e-06 1892.92783442644 -1632.25604110136;-0.00046 1.38580458351625e-06 1903.14609536116 -1620.33029517945;-0.00044 1.37578206788197e-06 1913.28922334674 -1608.34058139193;-0.00042 1.36570523872737e-06 1923.35681794986 -1596.28737307219;-0.0004 1.3555744938684e-06 1933.34848171912 -1584.17114606023;-0.00038 1.34539023324953e-06 1943.26382020074 -1571.99237868397;-0.00036 1.33515285892793e-06 1953.10244195415 -1559.75155174027;-0.00034 1.32486277505761e-06 1962.86395856739 -1547.44914847604;-0.00032 1.31452038787345e-06 1972.54798467251 -1535.08565456908;-0.0003 1.3041261056752e-06 1982.15413796074 -1522.66155810897;-0.00028 1.29368033881133e-06 1991.68203919759 -1510.17734957775;-0.00026 1.28318349966281e-06 2001.13131223785 -1497.63352183062;-0.00024 1.27263600262688e-06 2010.50158404038 -1485.0305700764;-0.00022 1.26203826410068e-06 2019.7924846829 -1472.36899185805;-0.0002 1.25139070246476e-06 2029.00364737657 -1459.64928703301;-0.00018 1.24069373806663e-06 2038.13470848044 -1446.87195775343;-0.00016 1.22994779320413e-06 2047.18530751588 -1434.0375084464;-0.00014 1.21915329210877e-06 2056.15508718071 -1421.14644579401;-0.00012 1.20831066092896e-06 2065.04369336341 -1408.19927871332;-0.0001 1.19742032771321e-06 2073.85077515701 -1395.19651833634;-8e-05 1.18648272239324e-06 2082.57598487301 -1382.13867798977;-6e-05 1.17549827676697e-06 2091.21897805507 -1369.0262731748;-4e-05 1.16446742448151e-06 2099.77941349261 -1355.8598215467;-2e-05 1.15339060101601e-06 2108.25695323431 -1342.63984289446]  x5=0.000530495096113056  V1=[8.92e-10 4.101e+05 4.101e+05;314.2 314.2 314.2;-0.7547 0.8912 -0.6796]  V2=[4.527e-10 4.161e+05 4.161e+05;314.2 314.2 314.2;-0.9521 0.7952 -0.7756]  I1=[5.472e-12 329.9 329.9;314.2 314.2 314.2;0.6215 -0.2451 -1.816]  I2=[4.185e-12 2499 2499;314.2 314.2 314.2;-1.63 0.9027 -0.6681]  nHarmo=1  Measurements=None  Decoupling=off  VsMag0=0  VrMag0=0  VsAngle0=0  VrAngle0=0  IsMag0=0  IrMag0=0  IsAngle0=0  IrAngle0=0
      settings: SourceProductBaseCode=PS
  Line_78_b : spsDistributedParametersLineLib/Distributed Parameters Line  Phases=3  Length=10  Frequency=50  Resistance=[0.0298 0.1619]  Inductance=[1.0568e-03 3.9470e-03]  Capacitance=[11.0414e-09 7.1301e-09]  x1=[-6e-05 -5.71138446100322e-05 0 0;-4e-05 -6.01239178751022e-05 323313.358785676 -261917.319610753;-2e-05 -6.31316175508431e-05 324952.630693455 -259880.7269496]  x2=[-6e-05 -4.51451515821985e-05 0 0;-4e-05 -4.80450121182784e-05 321258.852681484 -265289.90543446;-2e-05 -5.09429759195461e-05 322919.355584137 -263266.155098668]  x3=[-6e-05 -1.33994285532761e-06 0 0;-4e-05 -1.33686199413676e-06 -22.5571667684369 -328.404870477974;-2e-05 -1.33372835592346e-06 -20.4932982811499 -328.540127996714]  x4=[-6e-05 1.21324875676947e-06 0 0;-4e-05 1.20223023615616e-06 2095.38318770921 -1385.6461974489;-2e-05 1.19116425355167e-06 2104.04796597657 -1372.45325378746]  x5=5.30495096113055e-05  V1=[4.527e-10 4.161e+05 4.161e+05;314.2 314.2 314.2;-0.8021 0.8918 -0.679]  V2=[3.459e-10 4.166e+05 4.166e+05;314.2 314.2 314.2;-1.332 0.8824 -0.6884]  I1=[2.305e-11 329.2 329.2;314.2 314.2 314.2;1.554 -0.06674 -1.638]  I2=[1.894e-11 2512 2512;314.2 314.2 314.2;-2.04 0.9884 -0.5824]  nHarmo=1  Measurements=None  Decoupling=off  VsMag0=0  VrMag0=0  VsAngle0=0  VrAngle0=0  IsMag0=0  IrMag0=0  IsAngle0=0  IrAngle0=0
      settings: SourceProductBaseCode=PS
  Line_89_a : spsDistributedParametersLineLib/Distributed Parameters Line  Phases=3  Length=100  Frequency=50  Resistance=[0.0298 0.1619]  Inductance=[1.0568e-03 3.9470e-03]  Capacitance=[11.0414e-09 7.1301e-09]  x1=[-0.00054 2.46892450537955e-05 275804.124148785 -312280.917244423;-0.00052 2.1778254794557e-05 277760.776003612 -310541.839551969;-0.0005 1.88664047671096e-05 279706.462338606 -308790.502199423;-0.00048 1.59538099263065e-05 281641.1063414 -307026.974326584;-0.00046 1.30405852564048e-05 283564.631635562 -305251.325554513;-0.00044 1.01268457665262e-05 285476.962283609 -303463.625982783;-0.00042 7.21270648611668e-06 287378.022789999 -301663.946186712;-0.0004 4.29828246040522e-06 289267.738104119 -299852.357214577;-0.00038 1.38368874586208e-06 291146.033623245 -298028.930584809;-0.00036 -1.5309595943435e-06 293012.835195485 -296193.738283169;-0.00034 -4.44554749488572e-06 294868.069122709 -294346.852759906;-0.00032 -7.35995989282484e-06 296711.66216346 -292488.346926899;-0.0003 -1.02740817321497e-05 298543.541535841 -290618.294154775;-0.00028 -1.31877979683197e-05 300363.63492039 -288736.768270016;-0.00026 -1.61009935728071e-05 302171.870462937 -286843.843552043;-0.00024 -1.90135535376376e-05 303968.17677744 -284939.594730281;-0.00022 -2.19253628799309e-05 305752.4829488 -283024.096981214;-0.0002 -2.48363066464398e-05 307524.718535665 -281097.425925414;-0.00018 -2.77462699180889e-05 309284.81357321 -279159.657624553;-0.00016 -3.06551378145109e-05 311032.698575895 -277210.868578408;-0.00014 -3.3562795498582e-05 312768.304540213 -275251.135721832;-0.00012 -3.64691281809555e-05 314491.562947413 -273280.536421723;-0.0001 -3.93740211245936e-05 316202.405766204 -271299.148473968;-8e-05 -4.22773596492968e-05 317900.765455441 -269307.050100369;-6e-05 -4.51790291362315e-05 319586.574966791 -267304.31994556;-4e-05 -4.80789150324547e-05 321259.76774738 -265291.037073897;-2e-05 -5.09769028554368e-05 322920.277742425 -263267.280966342]  x2=[-0.00054 -0.000231405819033451 304427.901451653 -278456.804729767;-0.00052 -0.000233023918644757 306171.466326486 -276538.546679152;-0.0005 -0.000234632818870756 307902.944076078 -274609.371360224;-0.00048 -0.000236232456194821 309622.266344653 -272669.354933521;-0.00046 -0.000237822767466011 311329.36525631 -270718.57398757;-0.00044 -0.000239403689901559 313024.173417709 -268757.105535863;-0.00042 -0.000240975161089354 314706.623920724 -266785.027013815;-0.0004 -0.000242537118990405 316376.650345091 -264802.416275709;-0.00038 -0.000244089501941288 318034.186761026 -262809.351591624;-0.00036 -0.000245632248656583 319679.167731829 -260805.911644339;-0.00034 -0.000247165298231291 321311.528316468 -258792.175526234;-0.00032 -0.000248688590143239 322931.204072143 -256768.222736162;-0.0003 -0.000250202064255472 324538.131056828 -254734.133176314;-0.00028 -0.000251705660818622 326132.245831798 -252689.987149063;-0.00026 -0.000253199320473272 327713.485464129 -250635.865353794;-0.00024 -0.000254682984252297 329281.78752919 -248571.848883718;-0.00022 -0.00025615659358319 330837.0901131 -246498.019222671;-0.0002 -0.00025762009029038 332379.331815176 -244414.458241898;-0.00018 -0.00025907341659752 333908.451750357 -242321.248196818;-0.00016 -0.000260516515129779 335424.389551606 -240218.471723779;-0.00014 -0.000261949328916095 336927.085372293 -238106.211836797;-0.00012 -0.000263371801391435 338416.479888562 -235984.551924275;-0.0001 -0.000264783876399021 339892.514301666 -233853.575745712;-8e-05 -0.00026618549819255 341355.130340295 -231713.367428401;-6e-05 -0.000267576611438392 342804.270262872 -229564.011464101;-4e-05 -0.000268957161217779 344239.876859833 -227405.592705704;-2e-05 -0.00027032709302897 345661.89345589 -225238.196363889]  x3=[-0.00054 -1.79320257138823e-06 1915.22295481636 -1812.35176962715;-0.00052 -1.80836203717496e-06 1926.57236414964 -1800.28239086785;-0.0005 -1.82345011192488e-06 1937.8457157048 -1788.14194004234;-0.00048 -1.83846619998662e-06 1949.04256442923 -1775.93089643483;-0.00046 -1.85340970855075e-06 1960.16246829051 -1763.64974211641;-0.00044 -1.86828004767313e-06 1971.20498829388 -1751.29896192602;-0.00042 -1.88307663029823e-06 1982.16968849956 -1738.87904345131;-0.0004 -1.89779887228231e-06 1993.05613603995 -1726.39047700941;-0.00038 -1.91244619241647e-06 2003.86390113674 -1713.83375562753;-0.00036 -1.92701801244958e-06 2014.59255711789 -1701.20937502353;-0.00034 -1.94151375711115e-06 2025.24168043442 -1688.51783358635;-0.00032 -1.95593285413399e-06 2035.81085067717 -1675.75963235629;-0.0003 -1.97027473427684e-06 2046.2996505934 -1662.93527500532;-0.00028 -1.98453883134683e-06 2056.70766610325 -1650.04526781708;-0.00026 -1.99872458222183e-06 2067.0344863161 -1637.09011966701;-0.00024 -2.0128314268727e-06 2077.27970354675 -1624.07034200216;-0.00022 -2.02685880838535e-06 2087.44291333158 -1610.98644882105;-0.0002 -2.04080617298278e-06 2097.52371444447 -1597.8389566534;-0.00018 -2.05467297004693e-06 2107.52170891265 -1584.62838453968;-0.00016 -2.06845865214038e-06 2117.43650203241 -1571.35525401066;-0.00014 -2.08216267502801e-06 2127.26770238471 -1558.0200890668;-0.00012 -2.09578449769846e-06 2137.01492185058 -1544.62341615758;-0.0001 -2.10932358238551e-06 2146.67777562649 -1531.16576416071;-8e-05 -2.12277939458926e-06 2156.25588223952 -1517.64766436124;-6e-05 -2.13615140309729e-06 2165.74886356242 -1504.06965043062;-4e-05 -2.14943908000561e-06 2175.15634482855 -1490.43225840557;-2e-05 -2.16264190073948e-06 2184.47795464664 -1476.736026667]  x4=[-0.00054 1.59998827156172e-06 -155.291009896115 -183.601712293818;-0.00052 1.60901330875175e-06 -154.134359251666 -184.573810442025;-0.0005 1.61797482485143e-06 -152.971623646634 -185.538621932237;-0.00048 1.62687246607544e-06 -151.80284898383 -186.496108675348;-0.00046 1.63570588116015e-06 -150.628081404476 -187.446232871421;-0.00044 1.64447472137744e-06 -149.447367286384 -188.388957011179;-0.00042 1.65317864054852e-06 -148.260753242127 -189.324243877488;-0.0004 1.66181729505757e-06 -147.068286117196 -190.252056546824;-0.00038 1.6703903438653e-06 -145.870012988149 -191.172358390732;-0.00036 1.67889744852241e-06 -144.665981160759 -192.085113077269;-0.00034 1.687338273183e-06 -143.456238168141 -192.990284572445;-0.00032 1.69571248461774e-06 -142.240831768877 -193.887837141638;-0.0003 1.70401975222712e-06 -141.019809945129 -194.77773535101;-0.00028 1.71225974805443e-06 -139.79322090075 -195.659944068903;-0.00026 1.72043214679874e-06 -138.561113059373 -196.534428467227;-0.00024 1.72853662582775e-06 -137.323535062508 -197.401154022837;-0.00022 1.7365728651905e-06 -136.080535767614 -198.260086518891;-0.0002 1.74454054763002e-06 -134.832164246175 -199.111192046204;-0.00018 1.75243935859585e-06 -133.578469781761 -199.954437004589;-0.00016 1.76026898625646e-06 -132.319501868083 -200.789788104177;-0.00014 1.76802912151156e-06 -131.055310207039 -201.617212366739;-0.00012 1.77571945800429e-06 -129.785944706751 -202.43667712698;-0.0001 1.78333969213334e-06 -128.511455479594 -203.248150033835;-8e-05 1.79088952306491e-06 -127.231892840222 -204.051599051743;-6e-05 1.7983686527446e-06 -125.947307303577 -204.846992461913;-4e-05 1.80577678590918e-06 -124.657749582895 -205.634298863575;-2e-05 1.81311363009824e-06 -123.363270587709 -206.413487175221]  x5=0.000530495096113056  V1=[5.499e-10 4.166e+05 4.166e+05;314.2 314.2 314.2;-1.286 0.7858 -0.785]  V2=[5.945e-10 4.126e+05 4.126e+05;314.2 314.2 314.2;-0.5426 0.8923 -0.6785]  I1=[4.251e-12 2637 2637;314.2 314.2 314.2;-0.8207 0.8753 -0.6955]  I2=[3.147e-12 240.5 240.5;314.2 314.2 314.2;2.253 -0.6397 -2.211]  nHarmo=1  Measurements=None  Decoupling=off  VsMag0=0  VrMag0=0  VsAngle0=0  VrAngle0=0  IsMag0=0  IrMag0=0  IsAngle0=0  IrAngle0=0
      settings: SourceProductBaseCode=PS
  Line_89_b : spsDistributedParametersLineLib/Distributed Parameters Line  Phases=3  Length=10  Frequency=50  Resistance=[0.0298 0.1619]  Inductance=[1.0568e-03 3.9470e-03]  Capacitance=[11.0414e-09 7.1301e-09]  x1=[-6e-05 -0.000267576611644103 0 0;-4e-05 -0.000268957161354924 344239.876859833 -227405.592705704;-2e-05 -0.000270327093097544 345661.89345589 -225238.196363889]  x2=[-6e-05 -0.000289571452366695 0 0;-4e-05 -0.000290797026032151 346337.803657647 -223446.549527834;-2e-05 -0.000292011119528944 347734.903601703 -221266.049683916]  x3=[-6e-05 -2.53237651476569e-06 0 0;-4e-05 -2.54355357999829e-06 2346.58187224473 -1260.92249677741;-2e-05 -2.55463023009081e-06 2354.45805426627 -1246.15369817876]  x4=[-6e-05 1.78940495977015e-06 0 0;-4e-05 1.79704554501704e-06 -123.834725612585 -207.299524556174;-2e-05 1.80461518598286e-06 -122.529800102991 -208.073508972388]  x5=5.30495096113055e-05  V1=[5.916e-10 4.126e+05 4.126e+05;314.2 314.2 314.2;-0.4212 0.9888 -0.582]  V2=[6.139e-10 4.122e+05 4.122e+05;314.2 314.2 314.2;-0.1116 0.9997 -0.5711]  I1=[1.499e-11 2664 2664;314.2 314.2 314.2;1.83 1.08 -0.4912]  I2=[2.162e-11 241.5 241.5;314.2 314.2 314.2;2.618 -0.5367 -2.107]  nHarmo=1  Measurements=None  Decoupling=off  VsMag0=0  VrMag0=0  VsAngle0=0  VrAngle0=0  IsMag0=0  IrMag0=0  IsAngle0=0  IrAngle0=0
      settings: SourceProductBaseCode=PS
  Ln_45 : spsThreePhaseVIMeasurementLib/Three-Phase V-I Measurement  VoltageMeasurement=phase-to-ground  SetLabelV=on  LabelV=Vabc_Ln_45  Vpu=off  VpuLL=off  CurrentMeasurement=yes  SetLabelI=on  LabelI=Iabc_Ln_45  Ipu=off  Pbase=100e6  Vbase=500e3  OutputType=Complex  PhasorSimulation=off  PSBequivalent=0
  Ln_46 : spsThreePhaseVIMeasurementLib/Three-Phase V-I Measurement  VoltageMeasurement=phase-to-ground  SetLabelV=on  LabelV=Vabc_Ln_46  Vpu=off  VpuLL=off  CurrentMeasurement=yes  SetLabelI=on  LabelI=Iabc_Ln_46  Ipu=off  Pbase=100e6  Vbase=500e3  OutputType=Complex  PhasorSimulation=off  PSBequivalent=0
  Ln_54 : spsThreePhaseVIMeasurementLib/Three-Phase V-I Measurement  VoltageMeasurement=phase-to-ground  SetLabelV=on  LabelV=Vabc_Ln_54  Vpu=off  VpuLL=off  CurrentMeasurement=yes  SetLabelI=on  LabelI=Iabc_Ln_54  Ipu=off  Pbase=100e6  Vbase=500e3  OutputType=Complex  PhasorSimulation=off  PSBequivalent=0
  Ln_57 : spsThreePhaseVIMeasurementLib/Three-Phase V-I Measurement  VoltageMeasurement=phase-to-ground  SetLabelV=on  LabelV=Vabc_Ln_57  Vpu=off  VpuLL=off  CurrentMeasurement=yes  SetLabelI=on  LabelI=Iabc_Ln_57  Ipu=off  Pbase=100e6  Vbase=500e3  OutputType=Complex  PhasorSimulation=off  PSBequivalent=0
  Ln_64 : spsThreePhaseVIMeasurementLib/Three-Phase V-I Measurement  VoltageMeasurement=phase-to-ground  SetLabelV=on  LabelV=Vabc_Ln_64  Vpu=off  VpuLL=off  CurrentMeasurement=yes  SetLabelI=on  LabelI=Iabc_Ln_64  Ipu=off  Pbase=100e6  Vbase=500e3  OutputType=Complex  PhasorSimulation=off  PSBequivalent=0
  Ln_69 : spsThreePhaseVIMeasurementLib/Three-Phase V-I Measurement  VoltageMeasurement=phase-to-ground  SetLabelV=on  LabelV=Vabc_Ln_69  Vpu=off  VpuLL=off  CurrentMeasurement=yes  SetLabelI=on  LabelI=Iabc_Ln_69  Ipu=off  Pbase=100e6  Vbase=500e3  OutputType=Complex  PhasorSimulation=off  PSBequivalent=0
  Ln_75 : spsThreePhaseVIMeasurementLib/Three-Phase V-I Measurement  VoltageMeasurement=phase-to-ground  SetLabelV=on  LabelV=Vabc_Ln_75  Vpu=off  VpuLL=off  CurrentMeasurement=yes  SetLabelI=on  LabelI=Iabc_Ln_75  Ipu=off  Pbase=100e6  Vbase=500e3  OutputType=Complex  PhasorSimulation=off  PSBequivalent=0
  Ln_78 : spsThreePhaseVIMeasurementLib/Three-Phase V-I Measurement  VoltageMeasurement=phase-to-ground  SetLabelV=on  LabelV=Vabc_Ln_78  Vpu=off  VpuLL=off  CurrentMeasurement=yes  SetLabelI=on  LabelI=Iabc_Ln_78  Ipu=off  Pbase=100e6  Vbase=500e3  OutputType=Complex  PhasorSimulation=off  PSBequivalent=0
  Ln_87 : spsThreePhaseVIMeasurementLib/Three-Phase V-I Measurement  VoltageMeasurement=phase-to-ground  SetLabelV=on  LabelV=Vabc_Ln_87  Vpu=off  VpuLL=off  CurrentMeasurement=yes  SetLabelI=on  LabelI=Iabc_Ln_87  Ipu=off  Pbase=100e6  Vbase=500e3  OutputType=Complex  PhasorSimulation=off  PSBequivalent=0
  Ln_89 : spsThreePhaseVIMeasurementLib/Three-Phase V-I Measurement  VoltageMeasurement=phase-to-ground  SetLabelV=on  LabelV=Vabc_Ln_89  Vpu=off  VpuLL=off  CurrentMeasurement=yes  SetLabelI=on  LabelI=Iabc_Ln_89  Ipu=off  Pbase=100e6  Vbase=500e3  OutputType=Complex  PhasorSimulation=off  PSBequivalent=0
  Ln_96 : spsThreePhaseVIMeasurementLib/Three-Phase V-I Measurement  VoltageMeasurement=phase-to-ground  SetLabelV=on  LabelV=Vabc_Ln_96  Vpu=off  VpuLL=off  CurrentMeasurement=yes  SetLabelI=on  LabelI=Iabc_Ln_96  Ipu=off  Pbase=100e6  Vbase=500e3  OutputType=Complex  PhasorSimulation=off  PSBequivalent=0
  Ln_98 : spsThreePhaseVIMeasurementLib/Three-Phase V-I Measurement  VoltageMeasurement=phase-to-ground  SetLabelV=on  LabelV=Vabc_Ln_98  Vpu=off  VpuLL=off  CurrentMeasurement=yes  SetLabelI=on  LabelI=Iabc_Ln_98  Ipu=off  Pbase=100e6  Vbase=500e3  OutputType=Complex  PhasorSimulation=off  PSBequivalent=0
  "Load A 1020 MW, 320 MVAR" : spsThreePhaseParallelRLCLoadLib/Three-Phase Parallel RLC Load  LConnTagsString=A|B|C  Configuration=Y (grounded)  NominalVoltage=(400000)*1.04156  Vabc=[1e3 1e3 1e3]  Vabcp=[1e3 1e3 1e3]  NominalFrequency=50  UnbalancedPower=off  ActivePower=1020000000  InductivePower=320000000  CapacitivePower=0  Pabc=[10e3 9e3 11e3]  QLabc=[100 90 110]  QCabc=[100 90 110]  Pabcp=[10e3 9e3 11e3]  QLabcp=[100 90 110]  QCabcp=[100 90 110]  Measurements=None  LoadType=constant PQ
  "Load B 850 MW, 250 MVAR" : spsThreePhaseParallelRLCLoadLib/Three-Phase Parallel RLC Load  LConnTagsString=A|B|C  Configuration=Y (grounded)  NominalVoltage=(400000)*1.05046  Vabc=[1e3 1e3 1e3]  Vabcp=[1e3 1e3 1e3]  NominalFrequency=50  UnbalancedPower=off  ActivePower=850000000  InductivePower=280000000  CapacitivePower=0  Pabc=[10e3 9e3 11e3]  QLabc=[100 90 110]  QCabc=[100 90 110]  Pabcp=[10e3 9e3 11e3]  QLabcp=[100 90 110]  QCabcp=[100 90 110]  Measurements=None  LoadType=constant PQ
  "Load C 360 MW, 120 MVAR" : spsThreePhaseParallelRLCLoadLib/Three-Phase Parallel RLC Load  LConnTagsString=A|B|C  Configuration=Y (grounded)  NominalVoltage=(400000)*1.05886  Vabc=[1e3 1e3 1e3]  Vabcp=[1e3 1e3 1e3]  NominalFrequency=50  UnbalancedPower=off  ActivePower=360000000  InductivePower=120000000  CapacitivePower=0  Pabc=[10e3 9e3 11e3]  QLabc=[100 90 110]  QCabc=[100 90 110]  Pabcp=[10e3 9e3 11e3]  QLabcp=[100 90 110]  QCabcp=[100 90 110]  Measurements=None  LoadType=constant PQ
  Load Flow Bus : spsLoadFlowBusLib/Load Flow Bus  LConnTagsString=a  Phases=single  Connectors=on one side  ID=BUS_1  Vbase=24e3  Vref=1  Vangle=0  VLF=1  VLFb=1  VLFc=1  angleLF=0  angleLFb=0  angleLFc=0
      settings: SourceProductBaseCode=PS
  Load Flow Bus1 : spsLoadFlowBusLib/Load Flow Bus  LConnTagsString=a  Phases=single  Connectors=on one side  ID=BUS_4  Vbase=400e3  Vref=1  Vangle=0  VLF=1.038  VLFb=1  VLFc=1  angleLF=25.46  angleLFb=0  angleLFc=0
      settings: SourceProductBaseCode=PS
  Load Flow Bus2 : spsLoadFlowBusLib/Load Flow Bus  LConnTagsString=a  Phases=single  Connectors=on one side  ID=BUS_5  Vbase=400e3  Vref=1  Vangle=0  VLF=1.05  VLFb=1  VLFc=1  angleLF=20.03  angleLFb=0  angleLFc=0
      settings: SourceProductBaseCode=PS
  Load Flow Bus3 : spsLoadFlowBusLib/Load Flow Bus  LConnTagsString=a  Phases=single  Connectors=on one side  ID=BUS_2  Vbase=26e3  Vref=1  Vangle=0  VLF=1  VLFb=1  VLFc=1  angleLF=4.042  angleLFb=0  angleLFc=0
      settings: SourceProductBaseCode=PS
  Load Flow Bus4 : spsLoadFlowBusLib/Load Flow Bus  LConnTagsString=a  Phases=single  Connectors=on one side  ID=BUS_7  Vbase=400e3  Vref=1  Vangle=0  VLF=1.025  VLFb=1  VLFc=1  angleLF=27.21  angleLFb=0  angleLFc=0
      settings: SourceProductBaseCode=PS
  Load Flow Bus5 : spsLoadFlowBusLib/Load Flow Bus  LConnTagsString=a  Phases=single  Connectors=on one side  ID=BUS_8  Vbase=400e3  Vref=1  Vangle=0  VLF=1.042  VLFb=1  VLFc=1  angleLF=21.17  angleLFb=0  angleLFc=0
      settings: SourceProductBaseCode=PS
  Load Flow Bus6 : spsLoadFlowBusLib/Load Flow Bus  LConnTagsString=a  Phases=single  Connectors=on one side  ID=BUS_9  Vbase=400e3  Vref=1  Vangle=0  VLF=1.03  VLFb=1  VLFc=1  angleLF=27.89  angleLFb=0  angleLFc=0
      settings: SourceProductBaseCode=PS
  Load Flow Bus7 : spsLoadFlowBusLib/Load Flow Bus  LConnTagsString=a  Phases=single  Connectors=on one side  ID=BUS_3  Vbase=26e3  Vref=1  Vangle=0  VLF=1  VLFb=1  VLFc=1  angleLF=4.554  angleLFb=0  angleLFc=0
      settings: SourceProductBaseCode=PS
  Load Flow Bus8 : spsLoadFlowBusLib/Load Flow Bus  LConnTagsString=a  Phases=single  Connectors=on one side  ID=BUS_6  Vbase=400e3  Vref=1  Vangle=0  VLF=1.059  VLFb=1  VLFc=1  angleLF=23.91  angleLFb=0  angleLFc=0
      settings: SourceProductBaseCode=PS
  Power Balance : Subsystem  Commented=on
  Relay : Relay  OnSwitchValue=20
  Rotor Angle Deviations : Scope  NumInputPorts=2
  Scope : Scope  NumInputPorts=2
  Scope1 : Scope  NumInputPorts=3
  Shunt Compensation 200 MVAr : spsThreePhaseParallelRLCLoadLib/Three-Phase Parallel RLC Load  LConnTagsString=A|B|C  Configuration=Y (grounded)  NominalVoltage=(400000)*0.905282  Vabc=[1e3 1e3 1e3]  Vabcp=[1e3 1e3 1e3]  NominalFrequency=50  UnbalancedPower=off  ActivePower=0  InductivePower=0  CapacitivePower=200000000  Pabc=[10e3 9e3 11e3]  QLabc=[100 90 110]  QCabc=[100 90 110]  Pabcp=[10e3 9e3 11e3]  QLabcp=[100 90 110]  QCabcp=[100 90 110]  Measurements=None  LoadType=constant Z
  Shunt Compensation 350 MVAr : spsThreePhaseParallelRLCLoadLib/Three-Phase Parallel RLC Load  LConnTagsString=A|B|C  Configuration=Y (grounded)  NominalVoltage=(400000)*0.905282  Vabc=[1e3 1e3 1e3]  Vabcp=[1e3 1e3 1e3]  NominalFrequency=50  UnbalancedPower=off  ActivePower=0  InductivePower=0  CapacitivePower=350000000  Pabc=[10e3 9e3 11e3]  QLabc=[100 90 110]  QCabc=[100 90 110]  Pabcp=[10e3 9e3 11e3]  QLabcp=[100 90 110]  QCabcp=[100 90 110]  Measurements=None  LoadType=constant Z
  Shunt Compensation 400 MVAr : spsThreePhaseParallelRLCLoadLib/Three-Phase Parallel RLC Load  LConnTagsString=A|B|C  Configuration=Y (grounded)  NominalVoltage=(400000)*0.905282  Vabc=[1e3 1e3 1e3]  Vabcp=[1e3 1e3 1e3]  NominalFrequency=50  UnbalancedPower=off  ActivePower=0  InductivePower=0  CapacitivePower=400000000  Pabc=[10e3 9e3 11e3]  QLabc=[100 90 110]  QCabc=[100 90 110]  Pabcp=[10e3 9e3 11e3]  QLabcp=[100 90 110]  QCabcp=[100 90 110]  Measurements=None  LoadType=constant Z
  Snb_G1 : spsThreePhaseSeriesRLCLoadLib/Three-Phase Series RLC Load  LConnTagsString=A|B|C  Configuration=Y (grounded)  NominalVoltage=26e3  Vabc=[1e3 1e3 1e3]  Vabcp=[1e3 1e3 1e3]  NominalFrequency=50  UnbalancedPower=off  ActivePower=1000000  InductivePower=0  CapacitivePower=10000000  Pabc=[10e3 9e3 11e3]  QLabc=[100 90 110]  QCabc=[100 90 110]  Pabcp=[10e3 9e3 11e3]  QLabcp=[100 90 110]  QCabcp=[100 90 110]  Measurements=None  LoadType=constant Z
  Snb_G2 : spsThreePhaseSeriesRLCLoadLib/Three-Phase Series RLC Load  LConnTagsString=A|B|C  Configuration=Y (grounded)  NominalVoltage=26e3  Vabc=[1e3 1e3 1e3]  Vabcp=[1e3 1e3 1e3]  NominalFrequency=50  UnbalancedPower=off  ActivePower=1000000  InductivePower=0  CapacitivePower=10000000  Pabc=[10e3 9e3 11e3]  QLabc=[100 90 110]  QCabc=[100 90 110]  Pabcp=[10e3 9e3 11e3]  QLabcp=[100 90 110]  QCabcp=[100 90 110]  Measurements=None  LoadType=constant Z
  Snb_G3 : spsThreePhaseSeriesRLCLoadLib/Three-Phase Series RLC Load  LConnTagsString=A|B|C  Configuration=Y (grounded)  NominalVoltage=26e3  Vabc=[1e3 1e3 1e3]  Vabcp=[1e3 1e3 1e3]  NominalFrequency=50  UnbalancedPower=off  ActivePower=1000000  InductivePower=0  CapacitivePower=10000000  Pabc=[10e3 9e3 11e3]  QLabc=[100 90 110]  QCabc=[100 90 110]  Pabcp=[10e3 9e3 11e3]  QLabcp=[100 90 110]  QCabcp=[100 90 110]  Measurements=None  LoadType=constant Z
  Subsystem_75 : Subsystem
  Subsystem_78 : Subsystem
  Subsystem_87 : Subsystem
  Subtract : Sum  Inputs=+-
  Subtract1 : Sum  Inputs=+-
  Three-Phase Breaker10 : spsThreePhaseBreakerLib/Three-Phase Breaker  InitialState=closed  SwitchA=on  SwitchB=on  SwitchC=on  SwitchTimes=[(20+(4/50)) 501]  External=off  BreakerResistance=0.01  SnubberResistance=10e6  SnubberCapacitance=inf  Measurements=None
  Three-Phase Breaker{4..9,12..13} (8 alike) : spsThreePhaseBreakerLib/Three-Phase Breaker  InitialState=closed  SwitchA=on  SwitchB=on  SwitchC=on  SwitchTimes=[500 501]  External=off  BreakerResistance=0.01  SnubberResistance=10e6  SnubberCapacitance=inf  Measurements=None
  Three-Phase Fault1 : spsThreePhaseFaultLib/Three-Phase Fault  InitialStates=0  FaultA=on  FaultB=on  FaultC=on  GroundFault=on  SwitchTimes=[0.5 0.5+(10/50)]  External=off  SwitchStatus=NaN  FaultResistance=0.001  GroundResistance=0.01  SnubberResistance=1e6  SnubberCapacitance=inf  Measurements=None
  Xmer_1 800 MVA 24 kV /400 kV : spsThreePhaseTransformerTwoWindingsLib/Three-Phase Transformer (Two Windings)  Winding1Connection=Delta (D1)  Winding2Connection=Yg  CoreType=Three single-phase transformers  SetSaturation=off  Hysteresis=off  DataFile='hysteresis'  SetInitialFlux=off  Measurements=None  UNITS=pu  NominalPower=[ 800e6 50 ]  Winding1="[ 24e3 1e-6  0]"  Winding2=[ 400e3 1e-6 0.15]  Rm=500  Lm=500  L0=0.5  Saturation="[ 0,0  ;  0.005,1.2  ;  1.0,1.4 ]"  InitialFluxes=[ 0.8 , -0.8 , 0.7 ]  BreakLoop=off  DiscreteSolver=Trapezoidal iterative  DataType=off  TransfoNumber=0
  Xmer_2 1250 MVA 26 kV / 400 kV : spsThreePhaseTransformerTwoWindingsLib/Three-Phase Transformer (Two Windings)  Winding1Connection=Delta (D1)  Winding2Connection=Yg  CoreType=Three single-phase transformers  SetSaturation=off  Hysteresis=off  DataFile='hysteresis'  SetInitialFlux=off  Measurements=None  UNITS=pu  NominalPower=[ 1250e6 50 ]  Winding1="[ 26e3 1e-6  0]"  Winding2=[ 400e3 1e-6 0.15]  Rm=500  Lm=500  L0=0.5  Saturation="[ 0,0  ;  0.005,1.2  ;  1.0,1.4 ]"  InitialFluxes=[ 0.8 , -0.8 , 0.7 ]  BreakLoop=off  DiscreteSolver=Trapezoidal iterative  DataType=off  TransfoNumber=0
  Xmer_3 1000 MVA 26 kV / 400 kV : spsThreePhaseTransformerTwoWindingsLib/Three-Phase Transformer (Two Windings)  Winding1Connection=Delta (D1)  Winding2Connection=Yg  CoreType=Three single-phase transformers  SetSaturation=off  Hysteresis=off  DataFile='hysteresis'  SetInitialFlux=off  Measurements=None  UNITS=pu  NominalPower=[1000e6 50 ]  Winding1="[ 26e3 1e-6  0]"  Winding2=[ 400e3 1e-6 0.15]  Rm=500  Lm=500  L0=0.5  Saturation="[ 0,0  ;  0.005,1.2  ;  1.0,1.4 ]"  InitialFluxes=[ 0.8 , -0.8 , 0.7 ]  BreakLoop=off  DiscreteSolver=Trapezoidal iterative  DataType=off  TransfoNumber=0
  powergui : spspowerguiLib/powergui  Priority=2  SimulationMode=Discrete  SampleTime=20e-6  frequency=60  Iterations=50  frequencyindice=50  Pbase=100e6  ErrMax=0.0001  UnitsV=kV  UnitsW=MW  buscounter=0  FunctionMessages=off  echomessages=off  EnableUseOfTLC=off  CurrentSourceSwitches=off  DisableSnubberDevices=off  DisableRonSwitches=off  DisableVfSwitches=off  DisplayEquations=off  AutomaticDiscreteSolvers=off  SolverType=Tustin  Interpol=off  ExternalGateDelay=off  methode=off  Ts=100  x0status=blocks  SPID=on  SwTol=0  HookPort=off  NonlinearTolerance=1e-4  nMaxIteration=100  ContinueOnMaxIteration=off  RestoreLinks=warning  ResistiveCurrentMeasurement=off  Frange=logspace(0,3,50)  Ylog=off  Xlog=off  ShowGrid=off  save=off  variable=ZData  structure=0  ZoomFFT=on  StartTime=0.0  cycles=2  DisplayStyle=off  fundamental=60  FreqAxis=off  MaxFrequency=1000  frequencyindicesteady=1  RmsSteady=1  display=off
  tag scope: PSS=global
  wires:
  Subtract1/1 -> Gain/1
  Subtract/1 -> Gain1/1
  Gain/1 -> Rotor Angle Deviations/1
  Gain1/1 -> Rotor Angle Deviations/2
  Gain2/1 -> Scope1/1
  Gain3/1 -> Scope1/2
  Gain4/1 -> Scope1/3
  [dtheta_G2] -> Gain3/1, Subtract1/1
  [dtheta_G3] -> Gain4/1, Subtract/1
  [dtheta_G1] -> Gain2/1, Subtract1/2, Subtract/2
  Constant/1 -> [PSS]
  [Vabc_Ln_78] -> Demux/1
  [Iabc_Ln_78] -> Demux1/1
  Demux/1 -> Scope/1
  Demux1/1 -> Scope/2
  Relay/1 -> ?
  [Vabc_Ln_75] -> Subsystem_75/1(In1)
  [Iabc_Ln_75] -> Subsystem_75/2(In2)
  [Iabc_Ln_78] -> Subsystem_78/2(In2)
  [Vabc_Ln_78] -> Subsystem_78/1(In1)
  [Iabc_Ln_87] -> Subsystem_87/2(In2)
  [Vabc_Ln_87] -> Subsystem_87/1(In1)
  connections:
  B2/RConn2 -- Snb_G2/LConn2 -- Xmer_2 1250 MVA 26 kV / 400 kV/LConn2
  B2/RConn3 -- Snb_G2/LConn3 -- Xmer_2 1250 MVA 26 kV / 400 kV/LConn3
  B2/RConn1 -- Snb_G2/LConn1 -- Load Flow Bus3/LConn1 -- Xmer_2 1250 MVA 26 kV / 400 kV/LConn1
  Xmer_3 1000 MVA 26 kV / 400 kV/LConn3 -- Snb_G3/LConn3 -- B3/RConn3
  Xmer_3 1000 MVA 26 kV / 400 kV/LConn2 -- B3/RConn2 -- Snb_G3/LConn2
  Xmer_3 1000 MVA 26 kV / 400 kV/LConn1 -- B3/RConn1 -- Load Flow Bus7/LConn1 -- Snb_G3/LConn1
  B7/LConn2 -- Xmer_2 1250 MVA 26 kV / 400 kV/RConn2
  B7/LConn3 -- Xmer_2 1250 MVA 26 kV / 400 kV/RConn3
  "Gen_2 1200 MVA, 26 kV"/RConn1 -- B2/LConn1
  "Gen_2 1200 MVA, 26 kV"/RConn2 -- B2/LConn2
  "Gen_2 1200 MVA, 26 kV"/RConn3 -- B2/LConn3
  B7/LConn1 -- Xmer_2 1250 MVA 26 kV / 400 kV/RConn1
  Line_78_b/LConn1 -- Line_78_a/RConn1
  Line_78_b/LConn2 -- Line_78_a/RConn2
  Line_78_b/LConn3 -- Line_78_a/RConn3
  B9/LConn2 -- Xmer_3 1000 MVA 26 kV / 400 kV/RConn2
  B9/LConn1 -- Xmer_3 1000 MVA 26 kV / 400 kV/RConn1
  B9/LConn3 -- Xmer_3 1000 MVA 26 kV / 400 kV/RConn3
  B_78/LConn1 -- Ln_78/RConn1
  B_78/LConn2 -- Ln_78/RConn2
  B_78/LConn3 -- Ln_78/RConn3
  B_78/RConn1 -- Line_78_a/LConn1
  B_78/RConn2 -- Line_78_a/LConn2
  B_78/RConn3 -- Line_78_a/LConn3
  Line_78_b/RConn1 -- B_87/RConn1
  Line_78_b/RConn2 -- B_87/RConn2
  Line_78_b/RConn3 -- B_87/RConn3
  Ln_87/RConn1 -- B_87/LConn1
  Ln_87/RConn2 -- B_87/LConn2
  Ln_87/RConn3 -- B_87/LConn3
  Ln_78/LConn1 -- Load Flow Bus4/LConn1 -- B7/RConn1 -- Ln_75/LConn1
  Ln_78/LConn2 -- B7/RConn2 -- Ln_75/LConn2
  Ln_78/LConn3 -- Ln_75/LConn3 -- B7/RConn3
  Line_89_b/LConn1 -- Line_89_a/RConn1
  Three-Phase Breaker4/RConn2 -- Line_89_a/LConn2
  Line_89_b/LConn2 -- Line_89_a/RConn2
  Three-Phase Breaker4/RConn1 -- Line_89_a/LConn1
  Line_89_b/RConn1 -- Three-Phase Breaker5/RConn1
  Line_89_b/LConn3 -- Line_89_a/RConn3
  Three-Phase Breaker4/LConn1 -- Ln_89/RConn1
  Ln_98/RConn1 -- Three-Phase Breaker5/LConn1
  Three-Phase Breaker4/LConn2 -- Ln_89/RConn2
  Three-Phase Breaker4/LConn3 -- Ln_89/RConn3
  Line_89_b/RConn3 -- Three-Phase Breaker5/RConn3
  Ln_98/RConn2 -- Three-Phase Breaker5/LConn2
  Line_89_b/RConn2 -- Three-Phase Breaker5/RConn2
  Three-Phase Breaker4/RConn3 -- Line_89_a/LConn3
  Ln_98/RConn3 -- Three-Phase Breaker5/LConn3
  Ln_87/LConn1 -- B8/LConn1 -- Load Flow Bus5/LConn1 -- Shunt Compensation 400 MVAr/LConn1 -- Ln_89/LConn1
  Ln_87/LConn2 -- Shunt Compensation 400 MVAr/LConn2 -- Ln_89/LConn2 -- B8/LConn2
  Ln_87/LConn3 -- Shunt Compensation 400 MVAr/LConn3 -- B8/LConn3 -- Ln_89/LConn3
  Ln_98/LConn1 -- B9/RConn1 -- Load Flow Bus6/LConn1 -- Ln_96/LConn1
  Ln_98/LConn2 -- B9/RConn2 -- Ln_96/LConn2
  Ln_98/LConn3 -- Ln_96/LConn3 -- B9/RConn3
  B8/RConn1 -- "Load A 1020 MW, 320 MVAR"/LConn1
  B8/RConn2 -- "Load A 1020 MW, 320 MVAR"/LConn2
  B8/RConn3 -- "Load A 1020 MW, 320 MVAR"/LConn3
  B6/RConn3 -- "Load C 360 MW, 120 MVAR"/LConn3
  B6/RConn2 -- "Load C 360 MW, 120 MVAR"/LConn2
  B6/RConn1 -- "Load C 360 MW, 120 MVAR"/LConn1
  B5/RConn1 -- "Load B 850 MW, 250 MVAR"/LConn1
  B5/RConn2 -- "Load B 850 MW, 250 MVAR"/LConn2
  B5/RConn3 -- "Load B 850 MW, 250 MVAR"/LConn3
  Line_69_b/LConn1 -- Line_69_a/RConn1
  Three-Phase Breaker6/RConn2 -- Line_69_a/LConn2
  Line_69_b/LConn2 -- Line_69_a/RConn2
  Three-Phase Breaker6/RConn1 -- Line_69_a/LConn1
  Line_69_b/RConn1 -- Three-Phase Breaker7/RConn1
  Line_69_b/LConn3 -- Line_69_a/RConn3
  Three-Phase Breaker6/LConn1 -- Ln_69/RConn1
  Ln_96/RConn1 -- Three-Phase Breaker7/LConn1
  Three-Phase Breaker6/LConn2 -- Ln_69/RConn2
  Three-Phase Breaker6/LConn3 -- Ln_69/RConn3
  Line_69_b/RConn3 -- Three-Phase Breaker7/RConn3
  Ln_96/RConn2 -- Three-Phase Breaker7/LConn2
  Line_69_b/RConn2 -- Three-Phase Breaker7/RConn2
  Three-Phase Breaker6/RConn3 -- Line_69_a/LConn3
  Ln_96/RConn3 -- Three-Phase Breaker7/LConn3
  Ln_64/RConn3 -- Three-Phase Breaker9/LConn3
  Three-Phase Breaker8/RConn3 -- Line_46_a/LConn3
  Line_46_b/RConn2 -- Three-Phase Breaker9/RConn2
  Ln_64/RConn2 -- Three-Phase Breaker9/LConn2
  Three-Phase Breaker8/LConn2 -- Ln_46/RConn2
  Ln_64/RConn1 -- Three-Phase Breaker9/LConn1
  Line_46_b/LConn2 -- Line_46_a/RConn2
  Line_46_b/RConn3 -- Three-Phase Breaker9/RConn3
  Line_46_b/RConn1 -- Three-Phase Breaker9/RConn1
  Line_46_b/LConn3 -- Line_46_a/RConn3
  Three-Phase Breaker8/RConn2 -- Line_46_a/LConn2
  Three-Phase Breaker8/RConn1 -- Line_46_a/LConn1
  Three-Phase Breaker8/LConn1 -- Ln_46/RConn1
  Line_46_b/LConn1 -- Line_46_a/RConn1
  Three-Phase Breaker8/LConn3 -- Ln_46/RConn3
  Ln_69/LConn1 -- Shunt Compensation 200 MVAr/LConn1 -- B6/LConn1 -- Ln_64/LConn1 -- Load Flow Bus8/LConn1
  Ln_69/LConn2 -- Shunt Compensation 200 MVAr/LConn2 -- B6/LConn2 -- Ln_64/LConn2
  Ln_69/LConn3 -- B6/LConn3 -- Shunt Compensation 200 MVAr/LConn3 -- Ln_64/LConn3
  Ln_57/LConn1 -- B5/LConn1 -- Ln_54/LConn1 -- Shunt Compensation 350 MVAr/LConn1 -- Load Flow Bus2/LConn1
  Ln_57/LConn2 -- Shunt Compensation 350 MVAr/LConn2 -- B5/LConn2 -- Ln_54/LConn2
  Ln_57/LConn3 -- Shunt Compensation 350 MVAr/LConn3 -- B5/LConn3 -- Ln_54/LConn3
  Three-Phase Breaker12/LConn3 -- Ln_45/RConn3
  Line_45_b/LConn1 -- Line_45_a/RConn1
  Three-Phase Breaker12/RConn1 -- Line_45_a/LConn1
  Three-Phase Breaker12/LConn1 -- Ln_45/RConn1
  Line_45_b/LConn3 -- Line_45_a/RConn3
  Line_45_b/RConn1 -- Three-Phase Breaker13/RConn1
  Line_45_b/LConn2 -- Line_45_a/RConn2
  Ln_54/RConn1 -- Three-Phase Breaker13/LConn1
  Ln_54/RConn2 -- Three-Phase Breaker13/LConn2
  Line_45_b/RConn2 -- Three-Phase Breaker13/RConn2
  Three-Phase Breaker12/RConn3 -- Line_45_a/LConn3
  Ln_54/RConn3 -- Three-Phase Breaker13/LConn3
  Ln_75/RConn3 -- B_75/LConn3
  Three-Phase Breaker10/RConn3 -- Line_57_a/LConn3
  Line_57_b/RConn2 -- B_75/RConn2
  Ln_75/RConn2 -- B_75/LConn2
  Three-Phase Breaker12/LConn2 -- Ln_45/RConn2
  Line_45_b/RConn3 -- Three-Phase Breaker13/RConn3
  Three-Phase Breaker10/LConn2 -- Ln_57/RConn2
  Ln_75/RConn1 -- B_75/LConn1
  Three-Phase Breaker10/LConn1 -- Ln_57/RConn1
  Line_57_b/LConn2 -- Three-Phase Fault1/LConn2 -- Line_57_a/RConn2
  Line_57_b/RConn3 -- B_75/RConn3
  Line_57_b/RConn1 -- B_75/RConn1
  Line_57_b/LConn3 -- Three-Phase Fault1/LConn3 -- Line_57_a/RConn3
  Three-Phase Breaker10/RConn2 -- Line_57_a/LConn2
  Three-Phase Breaker10/RConn1 -- Line_57_a/LConn1
  Line_57_b/LConn1 -- Three-Phase Fault1/LConn1 -- Line_57_a/RConn1
  Three-Phase Breaker10/LConn3 -- Ln_57/RConn3
  Three-Phase Breaker12/RConn2 -- Line_45_a/LConn2
  Xmer_1 800 MVA 24 kV /400 kV/RConn1 -- B4/LConn1
  Xmer_1 800 MVA 24 kV /400 kV/RConn2 -- B4/LConn2
  Xmer_1 800 MVA 24 kV /400 kV/RConn3 -- B4/LConn3
  Gen_1 776.5 MVA 24 kV/RConn1 -- B1/LConn1
  Gen_1 776.5 MVA 24 kV/RConn2 -- B1/LConn2
  Gen_1 776.5 MVA 24 kV/RConn3 -- B1/LConn3
  B1/RConn1 -- Load Flow Bus/LConn1 -- Snb_G1/LConn1 -- Xmer_1 800 MVA 24 kV /400 kV/LConn1
  B1/RConn2 -- Snb_G1/LConn2 -- Xmer_1 800 MVA 24 kV /400 kV/LConn2
  B1/RConn3 -- Snb_G1/LConn3 -- Xmer_1 800 MVA 24 kV /400 kV/LConn3
  Ln_45/LConn1 -- Load Flow Bus1/LConn1 -- B4/RConn1 -- Ln_46/LConn1
  Ln_45/LConn2 -- Ln_46/LConn2 -- B4/RConn2
  Ln_45/LConn3 -- Ln_46/LConn3 -- B4/RConn3
  Gen_3 960 MVA 26 kV/RConn1 -- B3/LConn1
  Gen_3 960 MVA 26 kV/RConn2 -- B3/LConn2
  Gen_3 960 MVA 26 kV/RConn3 -- B3/LConn3
